simulink model "v2012_PF"  (Simulink 7.6)
(part 4 of 4)

  PQ86 : PMComponent  Tag=PSATblock  Description=Power Flow  PhysicalDomain=psatdomain  LeftPortType=p1  RightPortType=p1  LConnTagsString=__newl0  mask(PQ){p2_3q=[100  115], p4_5q=[0.5061 0.2587]*1.0722*0.0909, p6_7q=[1.2  0.8], p8q=off, p9q=on}
      mask prompts: p2_3q "Power and Voltage Ratings [MVA, kV]"; p4_5q "Active and Reactive Powers [p.u.  p.u.]"; p6_7q "Maximum and Minimum Allowable Voltage [p.u.   p.u.]"; p8q "Allow conversion to impendance for min or max voltage"; p9q "Connected"
      mask help:
      | This block defines a constant power load:
      |
      | P = Pcost.
      | Q = Qcost.
      mask CallbackString: |||fm_block|fm_block
      mask Display: plot([1 -0.5 -0.5 1],[0 0.866 -0.866 0])
  PQ9 : PMComponent  Tag=PSATblock  Description=Power Flow  PhysicalDomain=psatdomain  LeftPortType=p1  RightPortType=p1  LConnTagsString=__newl0  mask(PQ){p2_3q=[100 115], p4_5q=[2.2396 1.0847]*1.0722*0.25, p6_7q=[1.2  0.8], p8q=off, p9q=on}
      mask prompts: p2_3q "Power and Voltage Ratings [MVA, kV]"; p4_5q "Active and Reactive Powers [p.u.  p.u.]"; p6_7q "Maximum and Minimum Allowable Voltage [p.u.   p.u.]"; p8q "Allow conversion to impendance for min or max voltage"; p9q "Connected"
      mask help:
      | This block defines a constant power load:
      |
      | P = Pcost.
      | Q = Qcost.
      mask CallbackString: |||fm_block|fm_block
      mask Display: plot([1 -0.5 -0.5 1],[0 0.866 -0.866 0])
  PQ92 : PMComponent  Tag=PSATblock  Description=Power Flow  PhysicalDomain=psatdomain  LeftPortType=p1  RightPortType=p1  LConnTagsString=__newl0  mask(PQ){p2_3q=[100  115], p4_5q=[0.5061 0.2587]*1.0722*0.0909, p6_7q=[1.2  0.8], p8q=off, p9q=on}
      mask prompts: p2_3q "Power and Voltage Ratings [MVA, kV]"; p4_5q "Active and Reactive Powers [p.u.  p.u.]"; p6_7q "Maximum and Minimum Allowable Voltage [p.u.   p.u.]"; p8q "Allow conversion to impendance for min or max voltage"; p9q "Connected"
      mask help:
      | This block defines a constant power load:
      |
      | P = Pcost.
      | Q = Qcost.
      mask CallbackString: |||fm_block|fm_block
      mask Display: plot([1 -0.5 -0.5 1],[0 0.866 -0.866 0])
  PQ95 : PMComponent  Tag=PSATblock  Description=Power Flow  PhysicalDomain=psatdomain  LeftPortType=p1  RightPortType=p1  LConnTagsString=__newl0  mask(PQ){p2_3q=[100 115], p4_5q=[0.2898 0.2057]*1.0722*0.1667, p6_7q=[1.2  0.8], p8q=off, p9q=on}
      mask prompts: p2_3q "Power and Voltage Ratings [MVA, kV]"; p4_5q "Active and Reactive Powers [p.u.  p.u.]"; p6_7q "Maximum and Minimum Allowable Voltage [p.u.   p.u.]"; p8q "Allow conversion to impendance for min or max voltage"; p9q "Connected"
      mask help:
      | This block defines a constant power load:
      |
      | P = Pcost.
      | Q = Qcost.
      mask CallbackString: |||fm_block|fm_block
      mask Display: plot([1 -0.5 -0.5 1],[0 0.866 -0.866 0])
  PQ96 : PMComponent  Tag=PSATblock  Description=Power Flow  PhysicalDomain=psatdomain  LeftPortType=p1  RightPortType=p1  LConnTagsString=__newl0  mask(PQ){p2_3q=[100 115], p4_5q=[0.2898 0.2057]*1.0722*0.1667, p6_7q=[1.2  0.8], p8q=off, p9q=on}
      mask prompts: p2_3q "Power and Voltage Ratings [MVA, kV]"; p4_5q "Active and Reactive Powers [p.u.  p.u.]"; p6_7q "Maximum and Minimum Allowable Voltage [p.u.   p.u.]"; p8q "Allow conversion to impendance for min or max voltage"; p9q "Connected"
      mask help:
      | This block defines a constant power load:
      |
      | P = Pcost.
      | Q = Qcost.
      mask CallbackString: |||fm_block|fm_block
      mask Display: plot([1 -0.5 -0.5 1],[0 0.866 -0.866 0])
  PQ97 : PMComponent  Tag=PSATblock  Description=Power Flow  PhysicalDomain=psatdomain  LeftPortType=p1  RightPortType=p1  LConnTagsString=__newl0  mask(PQ){p2_3q=[100 115], p4_5q=[0.2898 0.2057]*1.0722*0.1667, p6_7q=[1.2  0.8], p8q=off, p9q=on}
      mask prompts: p2_3q "Power and Voltage Ratings [MVA, kV]"; p4_5q "Active and Reactive Powers [p.u.  p.u.]"; p6_7q "Maximum and Minimum Allowable Voltage [p.u.   p.u.]"; p8q "Allow conversion to impendance for min or max voltage"; p9q "Connected"
      mask help:
      | This block defines a constant power load:
      |
      | P = Pcost.
      | Q = Qcost.
      mask CallbackString: |||fm_block|fm_block
      mask Display: plot([1 -0.5 -0.5 1],[0 0.866 -0.866 0])
  PQ98 : PMComponent  Tag=PSATblock  Description=Power Flow  PhysicalDomain=psatdomain  LeftPortType=p1  RightPortType=p1  LConnTagsString=__newl0  mask(PQ){p2_3q=[100 115], p4_5q=[0.2898 0.2057]*1.0722*0.1667, p6_7q=[1.2  0.8], p8q=off, p9q=on}
      mask prompts: p2_3q "Power and Voltage Ratings [MVA, kV]"; p4_5q "Active and Reactive Powers [p.u.  p.u.]"; p6_7q "Maximum and Minimum Allowable Voltage [p.u.   p.u.]"; p8q "Allow conversion to impendance for min or max voltage"; p9q "Connected"
      mask help:
      | This block defines a constant power load:
      |
      | P = Pcost.
      | Q = Qcost.
      mask CallbackString: |||fm_block|fm_block
      mask Display: plot([1 -0.5 -0.5 1],[0 0.866 -0.866 0])
  PQ99 : PMComponent  Tag=PSATblock  Description=Power Flow  PhysicalDomain=psatdomain  LeftPortType=p1  RightPortType=p1  LConnTagsString=__newl0  mask(PQ){p2_3q=[100 115], p4_5q=[0.2898 0.2057]*1.0722*0.1667, p6_7q=[1.2  0.8], p8q=off, p9q=on}
      mask prompts: p2_3q "Power and Voltage Ratings [MVA, kV]"; p4_5q "Active and Reactive Powers [p.u.  p.u.]"; p6_7q "Maximum and Minimum Allowable Voltage [p.u.   p.u.]"; p8q "Allow conversion to impendance for min or max voltage"; p9q "Connected"
      mask help:
      | This block defines a constant power load:
      |
      | P = Pcost.
      | Q = Qcost.
      mask CallbackString: |||fm_block|fm_block
      mask Display: plot([1 -0.5 -0.5 1],[0 0.866 -0.866 0])
  PV : PMComponent  Tag=PSATblock  Description=Power Flow  PhysicalDomain=psatdomain  LeftPortType=p1  RightPortType=p1  RConnTagsString=__newr0  mask(PV){p2_3q=[100  115], p4q=2.6539+1.75, p5q=1.04, p6_7q=[0.8  -0.2], p8_9q=[1.1  0.9], p10q=1, p11q=on}
      mask prompts: p2_3q "Power and Voltage Ratings [MVA, kV]"; p4q "Active Power [p.u.]"; p5q "Voltage Magnitude [p.u.]"; p6_7q "Qmax and Qmin [p.u.  p.u.]"; p8_9q "Vmax and Vmin [p.u.  p.u.]"; p10q "Loss Participation Factor"; p11q "Connected"
      mask help:
      | This block defines a PV bus for load flow studies:
      |
      | P = Pcost.
      | V = Vdes.
      mask init:
      | [x,y] = fm_draw('circle');
      | [xp,yp] = fm_draw('P');
      mask CallbackString: ||||||fm_block
      mask Display:
      | plot(x,y)
      | color('blue')
      | plot(0.3*xp-0.35,0.6*yp,[0.1 0.3 0.5],[0.3 -0.3 0.3])
  PV1 : PMComponent  Tag=PSATblock  Description=Power Flow  PhysicalDomain=psatdomain  LeftPortType=p1  RightPortType=p1  RConnTagsString=__newr0  mask(PV){p2_3q=[100  115], p4q=5.6441*0.5, p5q=1.04, p6_7q=[0.8  -0.2], p8_9q=[1.1  0.9], p10q=1, p11q=on}
      mask prompts: p2_3q "Power and Voltage Ratings [MVA, kV]"; p4q "Active Power [p.u.]"; p5q "Voltage Magnitude [p.u.]"; p6_7q "Qmax and Qmin [p.u.  p.u.]"; p8_9q "Vmax and Vmin [p.u.  p.u.]"; p10q "Loss Participation Factor"; p11q "Connected"
      mask help:
      | This block defines a PV bus for load flow studies:
      |
      | P = Pcost.
      | V = Vdes.
      mask init:
      | [x,y] = fm_draw('circle');
      | [xp,yp] = fm_draw('P');
      mask CallbackString: ||||||fm_block
      mask Display:
      | plot(x,y)
      | color('blue')
      | plot(0.3*xp-0.35,0.6*yp,[0.1 0.3 0.5],[0.3 -0.3 0.3])
  PV10 : PMComponent  Tag=PSATblock  Description=Power Flow  PhysicalDomain=psatdomain  LeftPortType=p1  RightPortType=p1  RConnTagsString=__newr0  mask(PV){p2_3q=[100  138], p4q=10.4361, p5q=1.04, p6_7q=[0.8  -0.2], p8_9q=[1.1  0.9], p10q=1, p11q=on}
      mask prompts: p2_3q "Power and Voltage Ratings [MVA, kV]"; p4q "Active Power [p.u.]"; p5q "Voltage Magnitude [p.u.]"; p6_7q "Qmax and Qmin [p.u.  p.u.]"; p8_9q "Vmax and Vmin [p.u.  p.u.]"; p10q "Loss Participation Factor"; p11q "Connected"
      mask help:
      | This block defines a PV bus for load flow studies:
      |
      | P = Pcost.
      | V = Vdes.
      mask init:
      | [x,y] = fm_draw('circle');
      | [xp,yp] = fm_draw('P');
      mask CallbackString: ||||||fm_block
      mask Display:
      | plot(x,y)
      | color('blue')
      | plot(0.3*xp-0.35,0.6*yp,[0.1 0.3 0.5],[0.3 -0.3 0.3])
  PV11 : PMComponent  Tag=PSATblock  Description=Power Flow  PhysicalDomain=psatdomain  LeftPortType=p1  RightPortType=p1  RConnTagsString=__newr0  mask(PV){p2_3q=[100  400], p4q=13.1628, p5q=1.03, p6_7q=[0.8  -0.2], p8_9q=[1.1  0.9], p10q=1, p11q=on}
      mask prompts: p2_3q "Power and Voltage Ratings [MVA, kV]"; p4q "Active Power [p.u.]"; p5q "Voltage Magnitude [p.u.]"; p6_7q "Qmax and Qmin [p.u.  p.u.]"; p8_9q "Vmax and Vmin [p.u.  p.u.]"; p10q "Loss Participation Factor"; p11q "Connected"
      mask help:
      | This block defines a PV bus for load flow studies:
      |
      | P = Pcost.
      | V = Vdes.
      mask init:
      | [x,y] = fm_draw('circle');
      | [xp,yp] = fm_draw('P');
      mask CallbackString: ||||||fm_block
      mask Display:
      | plot(x,y)
      | color('blue')
      | plot(0.3*xp-0.35,0.6*yp,[0.1 0.3 0.5],[0.3 -0.3 0.3])
  PV12 : PMComponent  Tag=PSATblock  Description=Power Flow  PhysicalDomain=psatdomain  LeftPortType=p1  RightPortType=p1  RConnTagsString=__newr0  mask(PV){p2_3q=[100  230], p4q=2.9239, p5q=1.03, p6_7q=[0.8  -0.2], p8_9q=[1.1  0.9], p10q=1, p11q=on}
      mask prompts: p2_3q "Power and Voltage Ratings [MVA, kV]"; p4q "Active Power [p.u.]"; p5q "Voltage Magnitude [p.u.]"; p6_7q "Qmax and Qmin [p.u.  p.u.]"; p8_9q "Vmax and Vmin [p.u.  p.u.]"; p10q "Loss Participation Factor"; p11q "Connected"
      mask help:
      | This block defines a PV bus for load flow studies:
      |
      | P = Pcost.
      | V = Vdes.
      mask init:
      | [x,y] = fm_draw('circle');
      | [xp,yp] = fm_draw('P');
      mask CallbackString: ||||||fm_block
      mask Display:
      | plot(x,y)
      | color('blue')
      | plot(0.3*xp-0.35,0.6*yp,[0.1 0.3 0.5],[0.3 -0.3 0.3])
  PV13 : PMComponent  Tag=PSATblock  Description=Power Flow  PhysicalDomain=psatdomain  LeftPortType=p1  RightPortType=p1  RConnTagsString=__newr0  mask(PV){p2_3q=[100  230], p4q=2.1010+2.8, p5q=1.04, p6_7q=[0.8  -0.2], p8_9q=[1.1  0.9], p10q=1, p11q=on}
      mask prompts: p2_3q "Power and Voltage Ratings [MVA, kV]"; p4q "Active Power [p.u.]"; p5q "Voltage Magnitude [p.u.]"; p6_7q "Qmax and Qmin [p.u.  p.u.]"; p8_9q "Vmax and Vmin [p.u.  p.u.]"; p10q "Loss Participation Factor"; p11q "Connected"
      mask help:
      | This block defines a PV bus for load flow studies:
      |
      | P = Pcost.
      | V = Vdes.
      mask init:
      | [x,y] = fm_draw('circle');
      | [xp,yp] = fm_draw('P');
      mask CallbackString: ||||||fm_block
      mask Display:
      | plot(x,y)
      | color('blue')
      | plot(0.3*xp-0.35,0.6*yp,[0.1 0.3 0.5],[0.3 -0.3 0.3])
  PV14 : PMComponent  Tag=PSATblock  Description=Power Flow  PhysicalDomain=psatdomain  LeftPortType=p1  RightPortType=p1  RConnTagsString=__newr0  mask(PV){p2_3q=[100  400], p4q=14.6386, p5q=1.03, p6_7q=[0.8  -0.2], p8_9q=[1.1  0.9], p10q=1, p11q=on}
      mask prompts: p2_3q "Power and Voltage Ratings [MVA, kV]"; p4q "Active Power [p.u.]"; p5q "Voltage Magnitude [p.u.]"; p6_7q "Qmax and Qmin [p.u.  p.u.]"; p8_9q "Vmax and Vmin [p.u.  p.u.]"; p10q "Loss Participation Factor"; p11q "Connected"
      mask help:
      | This block defines a PV bus for load flow studies:
      |
      | P = Pcost.
      | V = Vdes.
      mask init:
      | [x,y] = fm_draw('circle');
      | [xp,yp] = fm_draw('P');
      mask CallbackString: ||||||fm_block
      mask Display:
      | plot(x,y)
      | color('blue')
      | plot(0.3*xp-0.35,0.6*yp,[0.1 0.3 0.5],[0.3 -0.3 0.3])
  PV15 : PMComponent  Tag=PSATblock  Description=Power Flow  PhysicalDomain=psatdomain  LeftPortType=p1  RightPortType=p1  RConnTagsString=__newr0  mask(PV){p2_3q=[100  230], p4q=5.04, p5q=1.02, p6_7q=[0.8  -0.2], p8_9q=[1.1  0.9], p10q=1, p11q=on}
      mask prompts: p2_3q "Power and Voltage Ratings [MVA, kV]"; p4q "Active Power [p.u.]"; p5q "Voltage Magnitude [p.u.]"; p6_7q "Qmax and Qmin [p.u.  p.u.]"; p8_9q "Vmax and Vmin [p.u.  p.u.]"; p10q "Loss Participation Factor"; p11q "Connected"
      mask help:
      | This block defines a PV bus for load flow studies:
      |
      | P = Pcost.
      | V = Vdes.
      mask init:
      | [x,y] = fm_draw('circle');
      | [xp,yp] = fm_draw('P');
      mask CallbackString: ||||||fm_block
      mask Display:
      | plot(x,y)
      | color('blue')
      | plot(0.3*xp-0.35,0.6*yp,[0.1 0.3 0.5],[0.3 -0.3 0.3])
  PV16 : PMComponent  Tag=PSATblock  Description=Power Flow  PhysicalDomain=psatdomain  LeftPortType=p1  RightPortType=p1  RConnTagsString=__newr0  mask(PV){p2_3q=[100  400], p4q=4.2*0.5, p5q=1.02, p6_7q=[0.8  -0.2], p8_9q=[1.1  0.9], p10q=1, p11q=on}
      mask prompts: p2_3q "Power and Voltage Ratings [MVA, kV]"; p4q "Active Power [p.u.]"; p5q "Voltage Magnitude [p.u.]"; p6_7q "Qmax and Qmin [p.u.  p.u.]"; p8_9q "Vmax and Vmin [p.u.  p.u.]"; p10q "Loss Participation Factor"; p11q "Connected"
      mask help:
      | This block defines a PV bus for load flow studies:
      |
      | P = Pcost.
      | V = Vdes.
      mask init:
      | [x,y] = fm_draw('circle');
      | [xp,yp] = fm_draw('P');
      mask CallbackString: ||||||fm_block
      mask Display:
      | plot(x,y)
      | color('blue')
      | plot(0.3*xp-0.35,0.6*yp,[0.1 0.3 0.5],[0.3 -0.3 0.3])
  PV17 : PMComponent  Tag=PSATblock  Description=Power Flow  PhysicalDomain=psatdomain  LeftPortType=p1  RightPortType=p1  RConnTagsString=__newr0  mask(PV){p2_3q=[100  400], p4q=4.2*0.5, p5q=1.02, p6_7q=[0.8  -0.2], p8_9q=[1.1  0.9], p10q=1, p11q=on}
      mask prompts: p2_3q "Power and Voltage Ratings [MVA, kV]"; p4q "Active Power [p.u.]"; p5q "Voltage Magnitude [p.u.]"; p6_7q "Qmax and Qmin [p.u.  p.u.]"; p8_9q "Vmax and Vmin [p.u.  p.u.]"; p10q "Loss Participation Factor"; p11q "Connected"
      mask help:
      | This block defines a PV bus for load flow studies:
      |
      | P = Pcost.
      | V = Vdes.
      mask init:
      | [x,y] = fm_draw('circle');
      | [xp,yp] = fm_draw('P');
      mask CallbackString: ||||||fm_block
      mask Display:
      | plot(x,y)
      | color('blue')
      | plot(0.3*xp-0.35,0.6*yp,[0.1 0.3 0.5],[0.3 -0.3 0.3])
  PV18 : PMComponent  Tag=PSATblock  Description=Power Flow  PhysicalDomain=psatdomain  LeftPortType=p1  RightPortType=p1  RConnTagsString=__newr0  mask(PV){p2_3q=[100  230], p4q=1.05, p5q=1.02, p6_7q=[0.8  -0.2], p8_9q=[1.1  0.9], p10q=1, p11q=on}
      mask prompts: p2_3q "Power and Voltage Ratings [MVA, kV]"; p4q "Active Power [p.u.]"; p5q "Voltage Magnitude [p.u.]"; p6_7q "Qmax and Qmin [p.u.  p.u.]"; p8_9q "Vmax and Vmin [p.u.  p.u.]"; p10q "Loss Participation Factor"; p11q "Connected"
      mask help:
      | This block defines a PV bus for load flow studies:
      |
      | P = Pcost.
      | V = Vdes.
      mask init:
      | [x,y] = fm_draw('circle');
      | [xp,yp] = fm_draw('P');
      mask CallbackString: ||||||fm_block
      mask Display:
      | plot(x,y)
      | color('blue')
      | plot(0.3*xp-0.35,0.6*yp,[0.1 0.3 0.5],[0.3 -0.3 0.3])
  PV19 : PMComponent  Tag=PSATblock  Description=Power Flow  PhysicalDomain=psatdomain  LeftPortType=p1  RightPortType=p1  RConnTagsString=__newr0  mask(PV){p2_3q=[100  230], p4q=2.997*0.5, p5q=1.02, p6_7q=[0.8  -0.2], p8_9q=[1.1  0.9], p10q=1, p11q=on}
      mask prompts: p2_3q "Power and Voltage Ratings [MVA, kV]"; p4q "Active Power [p.u.]"; p5q "Voltage Magnitude [p.u.]"; p6_7q "Qmax and Qmin [p.u.  p.u.]"; p8_9q "Vmax and Vmin [p.u.  p.u.]"; p10q "Loss Participation Factor"; p11q "Connected"
      mask help:
      | This block defines a PV bus for load flow studies:
      |
      | P = Pcost.
      | V = Vdes.
      mask init:
      | [x,y] = fm_draw('circle');
      | [xp,yp] = fm_draw('P');
      mask CallbackString: ||||||fm_block
      mask Display:
      | plot(x,y)
      | color('blue')
      | plot(0.3*xp-0.35,0.6*yp,[0.1 0.3 0.5],[0.3 -0.3 0.3])
  PV2 : PMComponent  Tag=PSATblock  Description=Power Flow  PhysicalDomain=psatdomain  LeftPortType=p1  RightPortType=p1  RConnTagsString=__newr0  mask(PV){p2_3q=[100  230], p4q=11.1020, p5q=1.04, p6_7q=[0.8  -0.2], p8_9q=[1.1  0.9], p10q=1, p11q=on}
      mask prompts: p2_3q "Power and Voltage Ratings [MVA, kV]"; p4q "Active Power [p.u.]"; p5q "Voltage Magnitude [p.u.]"; p6_7q "Qmax and Qmin [p.u.  p.u.]"; p8_9q "Vmax and Vmin [p.u.  p.u.]"; p10q "Loss Participation Factor"; p11q "Connected"
      mask help:
      | This block defines a PV bus for load flow studies:
      |
      | P = Pcost.
      | V = Vdes.
      mask init:
      | [x,y] = fm_draw('circle');
      | [xp,yp] = fm_draw('P');
      mask CallbackString: ||||||fm_block
      mask Display:
      | plot(x,y)
      | color('blue')
      | plot(0.3*xp-0.35,0.6*yp,[0.1 0.3 0.5],[0.3 -0.3 0.3])
  PV20 : PMComponent  Tag=PSATblock  Description=Power Flow  PhysicalDomain=psatdomain  LeftPortType=p1  RightPortType=p1  RConnTagsString=__newr0  mask(PV){p2_3q=[100  230], p4q=7.77, p5q=1.04, p6_7q=[0.8  -0.2], p8_9q=[1.1  0.9], p10q=1, p11q=on}
      mask prompts: p2_3q "Power and Voltage Ratings [MVA, kV]"; p4q "Active Power [p.u.]"; p5q "Voltage Magnitude [p.u.]"; p6_7q "Qmax and Qmin [p.u.  p.u.]"; p8_9q "Vmax and Vmin [p.u.  p.u.]"; p10q "Loss Participation Factor"; p11q "Connected"
      mask help:
      | This block defines a PV bus for load flow studies:
      |
      | P = Pcost.
      | V = Vdes.
      mask init:
      | [x,y] = fm_draw('circle');
      | [xp,yp] = fm_draw('P');
      mask CallbackString: ||||||fm_block
      mask Display:
      | plot(x,y)
      | color('blue')
      | plot(0.3*xp-0.35,0.6*yp,[0.1 0.3 0.5],[0.3 -0.3 0.3])
  PV21 : PMComponent  Tag=PSATblock  Description=Power Flow  PhysicalDomain=psatdomain  LeftPortType=p1  RightPortType=p1  RConnTagsString=__newr0  mask(PV){p2_3q=[100  115], p4q=0.4795, p5q=1.02, p6_7q=[0.8  -0.2], p8_9q=[1.1  0.9], p10q=1, p11q=on}
      mask prompts: p2_3q "Power and Voltage Ratings [MVA, kV]"; p4q "Active Power [p.u.]"; p5q "Voltage Magnitude [p.u.]"; p6_7q "Qmax and Qmin [p.u.  p.u.]"; p8_9q "Vmax and Vmin [p.u.  p.u.]"; p10q "Loss Participation Factor"; p11q "Connected"
      mask help:
      | This block defines a PV bus for load flow studies:
      |
      | P = Pcost.
      | V = Vdes.
      mask init:
      | [x,y] = fm_draw('circle');
      | [xp,yp] = fm_draw('P');
      mask CallbackString: ||||||fm_block
      mask Display:
      | plot(x,y)
      | color('blue')
      | plot(0.3*xp-0.35,0.6*yp,[0.1 0.3 0.5],[0.3 -0.3 0.3])
  PV22 : PMComponent  Tag=PSATblock  Description=Power Flow  PhysicalDomain=psatdomain  LeftPortType=p1  RightPortType=p1  RConnTagsString=__newr0  mask(PV){p2_3q=[100  230], p4q=1.1667, p5q=1.02, p6_7q=[0.8  -0.2], p8_9q=[1.1  0.9], p10q=1, p11q=on}
      mask prompts: p2_3q "Power and Voltage Ratings [MVA, kV]"; p4q "Active Power [p.u.]"; p5q "Voltage Magnitude [p.u.]"; p6_7q "Qmax and Qmin [p.u.  p.u.]"; p8_9q "Vmax and Vmin [p.u.  p.u.]"; p10q "Loss Participation Factor"; p11q "Connected"
      mask help:
      | This block defines a PV bus for load flow studies:
      |
      | P = Pcost.
      | V = Vdes.
      mask init:
      | [x,y] = fm_draw('circle');
      | [xp,yp] = fm_draw('P');
      mask CallbackString: ||||||fm_block
      mask Display:
      | plot(x,y)
      | color('blue')
      | plot(0.3*xp-0.35,0.6*yp,[0.1 0.3 0.5],[0.3 -0.3 0.3])
  PV23 : PMComponent  Tag=PSATblock  Description=Power Flow  PhysicalDomain=psatdomain  LeftPortType=p1  RightPortType=p1  RConnTagsString=__newr0  mask(PV){p2_3q=[100  115], p4q=4.2029*0.1, p5q=0.9833, p6_7q=[0.8  -0.2], p8_9q=[1.1  0.9], p10q=1, p11q=on}
      mask prompts: p2_3q "Power and Voltage Ratings [MVA, kV]"; p4q "Active Power [p.u.]"; p5q "Voltage Magnitude [p.u.]"; p6_7q "Qmax and Qmin [p.u.  p.u.]"; p8_9q "Vmax and Vmin [p.u.  p.u.]"; p10q "Loss Participation Factor"; p11q "Connected"
      mask help:
      | This block defines a PV bus for load flow studies:
      |
      | P = Pcost.
      | V = Vdes.
      mask init:
      | [x,y] = fm_draw('circle');
      | [xp,yp] = fm_draw('P');
      mask CallbackString: ||||||fm_block
      mask Display:
      | plot(x,y)
      | color('blue')
      | plot(0.3*xp-0.35,0.6*yp,[0.1 0.3 0.5],[0.3 -0.3 0.3])
  PV24 : PMComponent  Tag=PSATblock  Description=Power Flow  PhysicalDomain=psatdomain  LeftPortType=p1  RightPortType=p1  RConnTagsString=__newr0  mask(PV){p2_3q=[100  115], p4q=0.07, p5q=1.02, p6_7q=[0.8  -0.2], p8_9q=[1.1  0.9], p10q=1, p11q=on}
      mask prompts: p2_3q "Power and Voltage Ratings [MVA, kV]"; p4q "Active Power [p.u.]"; p5q "Voltage Magnitude [p.u.]"; p6_7q "Qmax and Qmin [p.u.  p.u.]"; p8_9q "Vmax and Vmin [p.u.  p.u.]"; p10q "Loss Participation Factor"; p11q "Connected"
      mask help:
      | This block defines a PV bus for load flow studies:
      |
      | P = Pcost.
      | V = Vdes.
      mask init:
      | [x,y] = fm_draw('circle');
      | [xp,yp] = fm_draw('P');
      mask CallbackString: ||||||fm_block
      mask Display:
      | plot(x,y)
      | color('blue')
      | plot(0.3*xp-0.35,0.6*yp,[0.1 0.3 0.5],[0.3 -0.3 0.3])
  PV25 : PMComponent  Tag=PSATblock  Description=Power Flow  PhysicalDomain=psatdomain  LeftPortType=p1  RightPortType=p1  RConnTagsString=__newr0  mask(PV){p2_3q=[100  115], p4q=2.8610*0.5, p5q=1.04, p6_7q=[0.8  -0.2], p8_9q=[1.1  0.9], p10q=1, p11q=on}
      mask prompts: p2_3q "Power and Voltage Ratings [MVA, kV]"; p4q "Active Power [p.u.]"; p5q "Voltage Magnitude [p.u.]"; p6_7q "Qmax and Qmin [p.u.  p.u.]"; p8_9q "Vmax and Vmin [p.u.  p.u.]"; p10q "Loss Participation Factor"; p11q "Connected"
      mask help:
      | This block defines a PV bus for load flow studies:
      |
      | P = Pcost.
      | V = Vdes.
      mask init:
      | [x,y] = fm_draw('circle');
      | [xp,yp] = fm_draw('P');
      mask CallbackString: ||||||fm_block
      mask Display:
      | plot(x,y)
      | color('blue')
      | plot(0.3*xp-0.35,0.6*yp,[0.1 0.3 0.5],[0.3 -0.3 0.3])
  PV26 : PMComponent  Tag=PSATblock  Description=Power Flow  PhysicalDomain=psatdomain  LeftPortType=p1  RightPortType=p1  RConnTagsString=__newr0  mask(PV){p2_3q=[100  115], p4q=0.6832, p5q=1.04, p6_7q=[0.8  -0.2], p8_9q=[1.1  0.9], p10q=1, p11q=on}
      mask prompts: p2_3q "Power and Voltage Ratings [MVA, kV]"; p4q "Active Power [p.u.]"; p5q "Voltage Magnitude [p.u.]"; p6_7q "Qmax and Qmin [p.u.  p.u.]"; p8_9q "Vmax and Vmin [p.u.  p.u.]"; p10q "Loss Participation Factor"; p11q "Connected"
      mask help:
      | This block defines a PV bus for load flow studies:
      |
      | P = Pcost.
      | V = Vdes.
      mask init:
      | [x,y] = fm_draw('circle');
      | [xp,yp] = fm_draw('P');
      mask CallbackString: ||||||fm_block
      mask Display:
      | plot(x,y)
      | color('blue')
      | plot(0.3*xp-0.35,0.6*yp,[0.1 0.3 0.5],[0.3 -0.3 0.3])
  PV27 : PMComponent  Tag=PSATblock  Description=Power Flow  PhysicalDomain=psatdomain  LeftPortType=p1  RightPortType=p1  RConnTagsString=__newr0  mask(PV){p2_3q=[100  115], p4q=1.8298, p5q=1.02, p6_7q=[0.8  -0.2], p8_9q=[1.1  0.9], p10q=1, p11q=on}
      mask prompts: p2_3q "Power and Voltage Ratings [MVA, kV]"; p4q "Active Power [p.u.]"; p5q "Voltage Magnitude [p.u.]"; p6_7q "Qmax and Qmin [p.u.  p.u.]"; p8_9q "Vmax and Vmin [p.u.  p.u.]"; p10q "Loss Participation Factor"; p11q "Connected"
      mask help:
      | This block defines a PV bus for load flow studies:
      |
      | P = Pcost.
      | V = Vdes.
      mask init:
      | [x,y] = fm_draw('circle');
      | [xp,yp] = fm_draw('P');
      mask CallbackString: ||||||fm_block
      mask Display:
      | plot(x,y)
      | color('blue')
      | plot(0.3*xp-0.35,0.6*yp,[0.1 0.3 0.5],[0.3 -0.3 0.3])
  PV28 : PMComponent  Tag=PSATblock  Description=Power Flow  PhysicalDomain=psatdomain  LeftPortType=p1  RightPortType=p1  RConnTagsString=__newr0  mask(PV){p2_3q=[100  115], p4q=4.1668*0.1, p5q=0.9513, p6_7q=[0.8  -0.2], p8_9q=[1.1  0.9], p10q=1, p11q=on}
      mask prompts: p2_3q "Power and Voltage Ratings [MVA, kV]"; p4q "Active Power [p.u.]"; p5q "Voltage Magnitude [p.u.]"; p6_7q "Qmax and Qmin [p.u.  p.u.]"; p8_9q "Vmax and Vmin [p.u.  p.u.]"; p10q "Loss Participation Factor"; p11q "Connected"
      mask help:
      | This block defines a PV bus for load flow studies:
      |
      | P = Pcost.
      | V = Vdes.
      mask init:
      | [x,y] = fm_draw('circle');
      | [xp,yp] = fm_draw('P');
      mask CallbackString: ||||||fm_block
      mask Display:
      | plot(x,y)
      | color('blue')
      | plot(0.3*xp-0.35,0.6*yp,[0.1 0.3 0.5],[0.3 -0.3 0.3])
  PV29 : PMComponent  Tag=PSATblock  Description=Power Flow  PhysicalDomain=psatdomain  LeftPortType=p1  RightPortType=p1  RConnTagsString=__newr0  mask(PV){p2_3q=[100  115], p4q=0.1499, p5q=1.02, p6_7q=[0.8  -0.2], p8_9q=[1.1  0.9], p10q=1, p11q=on}
      mask prompts: p2_3q "Power and Voltage Ratings [MVA, kV]"; p4q "Active Power [p.u.]"; p5q "Voltage Magnitude [p.u.]"; p6_7q "Qmax and Qmin [p.u.  p.u.]"; p8_9q "Vmax and Vmin [p.u.  p.u.]"; p10q "Loss Participation Factor"; p11q "Connected"
      mask help:
      | This block defines a PV bus for load flow studies:
      |
      | P = Pcost.
      | V = Vdes.
      mask init:
      | [x,y] = fm_draw('circle');
      | [xp,yp] = fm_draw('P');
      mask CallbackString: ||||||fm_block
      mask Display:
      | plot(x,y)
      | color('blue')
      | plot(0.3*xp-0.35,0.6*yp,[0.1 0.3 0.5],[0.3 -0.3 0.3])
  PV3 : PMComponent  Tag=PSATblock  Description=Power Flow  PhysicalDomain=psatdomain  LeftPortType=p1  RightPortType=p1  RConnTagsString=__newr0  mask(PV){p2_3q=[100  230], p4q=2.8610*0.5, p5q=1.04, p6_7q=[0.8  -0.2], p8_9q=[1.1  0.9], p10q=1, p11q=on}
      mask prompts: p2_3q "Power and Voltage Ratings [MVA, kV]"; p4q "Active Power [p.u.]"; p5q "Voltage Magnitude [p.u.]"; p6_7q "Qmax and Qmin [p.u.  p.u.]"; p8_9q "Vmax and Vmin [p.u.  p.u.]"; p10q "Loss Participation Factor"; p11q "Connected"
      mask help:
      | This block defines a PV bus for load flow studies:
      |
      | P = Pcost.
      | V = Vdes.
      mask init:
      | [x,y] = fm_draw('circle');
      | [xp,yp] = fm_draw('P');
      mask CallbackString: ||||||fm_block
      mask Display:
      | plot(x,y)
      | color('blue')
      | plot(0.3*xp-0.35,0.6*yp,[0.1 0.3 0.5],[0.3 -0.3 0.3])
  PV30 : PMComponent  Tag=PSATblock  Description=Power Flow  PhysicalDomain=psatdomain  LeftPortType=p1  RightPortType=p1  RConnTagsString=__newr0  mask(PV){p2_3q=[100  115], p4q=0.28, p5q=1.02, p6_7q=[0.8  -0.2], p8_9q=[1.1  0.9], p10q=1, p11q=on}
      mask prompts: p2_3q "Power and Voltage Ratings [MVA, kV]"; p4q "Active Power [p.u.]"; p5q "Voltage Magnitude [p.u.]"; p6_7q "Qmax and Qmin [p.u.  p.u.]"; p8_9q "Vmax and Vmin [p.u.  p.u.]"; p10q "Loss Participation Factor"; p11q "Connected"
      mask help:
      | This block defines a PV bus for load flow studies:
      |
      | P = Pcost.
      | V = Vdes.
      mask init:
      | [x,y] = fm_draw('circle');
      | [xp,yp] = fm_draw('P');
      mask CallbackString: ||||||fm_block
      mask Display:
      | plot(x,y)
      | color('blue')
      | plot(0.3*xp-0.35,0.6*yp,[0.1 0.3 0.5],[0.3 -0.3 0.3])
  PV38 : PMComponent  Tag=PSATblock  Description=Power Flow  PhysicalDomain=psatdomain  LeftPortType=p1  RightPortType=p1  RConnTagsString=__newr0  mask(PV){p2_3q=[100  115], p4q=5.6441*0.5, p5q=1.04, p6_7q=[0.8  -0.2], p8_9q=[1.1  0.9], p10q=1, p11q=on}
      mask prompts: p2_3q "Power and Voltage Ratings [MVA, kV]"; p4q "Active Power [p.u.]"; p5q "Voltage Magnitude [p.u.]"; p6_7q "Qmax and Qmin [p.u.  p.u.]"; p8_9q "Vmax and Vmin [p.u.  p.u.]"; p10q "Loss Participation Factor"; p11q "Connected"
      mask help:
      | This block defines a PV bus for load flow studies:
      |
      | P = Pcost.
      | V = Vdes.
      mask init:
      | [x,y] = fm_draw('circle');
      | [xp,yp] = fm_draw('P');
      mask CallbackString: ||||||fm_block
      mask Display:
      | plot(x,y)
      | color('blue')
      | plot(0.3*xp-0.35,0.6*yp,[0.1 0.3 0.5],[0.3 -0.3 0.3])
  PV4 : PMComponent  Tag=PSATblock  Description=Power Flow  PhysicalDomain=psatdomain  LeftPortType=p1  RightPortType=p1  RConnTagsString=__newr0  mask(PV){p2_3q=[100  230], p4q=1.7982, p5q=1.02, p6_7q=[0.8  -0.2], p8_9q=[1.1  0.9], p10q=1, p11q=on}
      mask prompts: p2_3q "Power and Voltage Ratings [MVA, kV]"; p4q "Active Power [p.u.]"; p5q "Voltage Magnitude [p.u.]"; p6_7q "Qmax and Qmin [p.u.  p.u.]"; p8_9q "Vmax and Vmin [p.u.  p.u.]"; p10q "Loss Participation Factor"; p11q "Connected"
      mask help:
      | This block defines a PV bus for load flow studies:
      |
      | P = Pcost.
      | V = Vdes.
      mask init:
      | [x,y] = fm_draw('circle');
      | [xp,yp] = fm_draw('P');
      mask CallbackString: ||||||fm_block
      mask Display:
      | plot(x,y)
      | color('blue')
      | plot(0.3*xp-0.35,0.6*yp,[0.1 0.3 0.5],[0.3 -0.3 0.3])
  PV5 : PMComponent  Tag=PSATblock  Description=Power Flow  PhysicalDomain=psatdomain  LeftPortType=p1  RightPortType=p1  RConnTagsString=__newr0  mask(PV){p2_3q=[100  138], p4q=4.62, p5q=1.04, p6_7q=[0.8  -0.2], p8_9q=[1.1  0.9], p10q=1, p11q=on}
      mask prompts: p2_3q "Power and Voltage Ratings [MVA, kV]"; p4q "Active Power [p.u.]"; p5q "Voltage Magnitude [p.u.]"; p6_7q "Qmax and Qmin [p.u.  p.u.]"; p8_9q "Vmax and Vmin [p.u.  p.u.]"; p10q "Loss Participation Factor"; p11q "Connected"
      mask help:
      | This block defines a PV bus for load flow studies:
      |
      | P = Pcost.
      | V = Vdes.
      mask init:
      | [x,y] = fm_draw('circle');
      | [xp,yp] = fm_draw('P');
      mask CallbackString: ||||||fm_block
      mask Display:
      | plot(x,y)
      | color('blue')
      | plot(0.3*xp-0.35,0.6*yp,[0.1 0.3 0.5],[0.3 -0.3 0.3])
  PV6 : PMComponent  Tag=PSATblock  Description=Power Flow  PhysicalDomain=psatdomain  LeftPortType=p1  RightPortType=p1  RConnTagsString=__newr0  mask(PV){p2_3q=[100  230], p4q=2.6539+4.83, p5q=1.02, p6_7q=[0.8  -0.2], p8_9q=[1.1  0.9], p10q=1, p11q=on}
      mask prompts: p2_3q "Power and Voltage Ratings [MVA, kV]"; p4q "Active Power [p.u.]"; p5q "Voltage Magnitude [p.u.]"; p6_7q "Qmax and Qmin [p.u.  p.u.]"; p8_9q "Vmax and Vmin [p.u.  p.u.]"; p10q "Loss Participation Factor"; p11q "Connected"
      mask help:
      | This block defines a PV bus for load flow studies:
      |
      | P = Pcost.
      | V = Vdes.
      mask init:
      | [x,y] = fm_draw('circle');
      | [xp,yp] = fm_draw('P');
      mask CallbackString: ||||||fm_block
      mask Display:
      | plot(x,y)
      | color('blue')
      | plot(0.3*xp-0.35,0.6*yp,[0.1 0.3 0.5],[0.3 -0.3 0.3])
  PV7 : PMComponent  Tag=PSATblock  Description=Power Flow  PhysicalDomain=psatdomain  LeftPortType=p1  RightPortType=p1  RConnTagsString=__newr0  mask(PV){p2_3q=[100  400], p4q=11.7691, p5q=1.04, p6_7q=[0.8  -0.2], p8_9q=[1.1  0.9], p10q=1, p11q=on}
      mask prompts: p2_3q "Power and Voltage Ratings [MVA, kV]"; p4q "Active Power [p.u.]"; p5q "Voltage Magnitude [p.u.]"; p6_7q "Qmax and Qmin [p.u.  p.u.]"; p8_9q "Vmax and Vmin [p.u.  p.u.]"; p10q "Loss Participation Factor"; p11q "Connected"
      mask help:
      | This block defines a PV bus for load flow studies:
      |
      | P = Pcost.
      | V = Vdes.
      mask init:
      | [x,y] = fm_draw('circle');
      | [xp,yp] = fm_draw('P');
      mask CallbackString: ||||||fm_block
      mask Display:
      | plot(x,y)
      | color('blue')
      | plot(0.3*xp-0.35,0.6*yp,[0.1 0.3 0.5],[0.3 -0.3 0.3])
  PV8 : PMComponent  Tag=PSATblock  Description=Power Flow  PhysicalDomain=psatdomain  LeftPortType=p1  RightPortType=p1  RConnTagsString=__newr0  mask(PV){p2_3q=[100  230], p4q=3.2368, p5q=1.04, p6_7q=[0.8  -0.2], p8_9q=[1.1  0.9], p10q=1, p11q=on}
      mask prompts: p2_3q "Power and Voltage Ratings [MVA, kV]"; p4q "Active Power [p.u.]"; p5q "Voltage Magnitude [p.u.]"; p6_7q "Qmax and Qmin [p.u.  p.u.]"; p8_9q "Vmax and Vmin [p.u.  p.u.]"; p10q "Loss Participation Factor"; p11q "Connected"
      mask help:
      | This block defines a PV bus for load flow studies:
      |
      | P = Pcost.
      | V = Vdes.
      mask init:
      | [x,y] = fm_draw('circle');
      | [xp,yp] = fm_draw('P');
      mask CallbackString: ||||||fm_block
      mask Display:
      | plot(x,y)
      | color('blue')
      | plot(0.3*xp-0.35,0.6*yp,[0.1 0.3 0.5],[0.3 -0.3 0.3])
  PV9 : PMComponent  Tag=PSATblock  Description=Power Flow  PhysicalDomain=psatdomain  LeftPortType=p1  RightPortType=p1  RConnTagsString=__newr0  mask(PV){p2_3q=[100  400], p4q=13.5944, p5q=1.04, p6_7q=[0.8  -0.2], p8_9q=[1.1  0.9], p10q=1, p11q=on}
      mask prompts: p2_3q "Power and Voltage Ratings [MVA, kV]"; p4q "Active Power [p.u.]"; p5q "Voltage Magnitude [p.u.]"; p6_7q "Qmax and Qmin [p.u.  p.u.]"; p8_9q "Vmax and Vmin [p.u.  p.u.]"; p10q "Loss Participation Factor"; p11q "Connected"
      mask help:
      | This block defines a PV bus for load flow studies:
      |
      | P = Pcost.
      | V = Vdes.
      mask init:
      | [x,y] = fm_draw('circle');
      | [xp,yp] = fm_draw('P');
      mask CallbackString: ||||||fm_block
      mask Display:
      | plot(x,y)
      | color('blue')
      | plot(0.3*xp-0.35,0.6*yp,[0.1 0.3 0.5],[0.3 -0.3 0.3])
  Palital 400kV : PMComponent  Tag=PSATblock  Description=Connection  PhysicalDomain=psatdomain  LeftPortType=p1  RightPortType=p1  LConnTagsString=__newl0|__newl1|__newl2  RConnTagsString=__newr0|__newr1  mask(Bus){in=3, out=2, p2q=400, p3_4q=[1.0189    -0.15846], p5q=1, p6q=1}
      mask prompts: in "Number of inputs:"; out "Number of outputs:"; p2q "Voltage Rating [kV]"; p3_4q "Voltage initial guess [p.u.  rad]"; p5q "Area number"; p6q "Region number"
      mask help: Bus block.
      mask init:
      | fm_inout
      settings: AttributesFormatString="|V| =  1.0017 p.u.\\n<V  = -0.1078 rad"
      mask CallbackString: ||||fm_block|
      mask Display: plot([0 1 1 0 0],[0 0 1 1 0])
  Palo Grande : PMComponent  Tag=PSATblock  Description=Connection  PhysicalDomain=psatdomain  LeftPortType=p1  RightPortType=p1  LConnTagsString=__newl0  RConnTagsString=__newr0|__newr1  mask(Bus){in=1, out=2, p2q=115, p3_4q=[1.0023    -0.25717], p5q=1, p6q=1}
      mask prompts: in "Number of inputs:"; out "Number of outputs:"; p2q "Voltage Rating [kV]"; p3_4q "Voltage initial guess [p.u.  rad]"; p5q "Area number"; p6q "Region number"
      mask help: Bus block.
      mask init:
      | fm_inout
      settings: AttributesFormatString="|V| =  1.0139 p.u.\\n<V  =  0.4686 rad"
      mask CallbackString: ||||fm_block|
      mask Display: plot([0 1 1 0 0],[0 0 1 1 0])
  Papelon 230kV : PMComponent  Tag=PSATblock  Description=Connection  PhysicalDomain=psatdomain  LeftPortType=p1  RightPortType=p1  LConnTagsString=__newl0|__newl1  RConnTagsString=__newr0|__newr1|__newr2  mask(Bus){in=2, out=3, p2q=230, p3_4q=[0.99933     -0.4575], p5q=1, p6q=1}
      mask prompts: in "Number of inputs:"; out "Number of outputs:"; p2q "Voltage Rating [kV]"; p3_4q "Voltage initial guess [p.u.  rad]"; p5q "Area number"; p6q "Region number"
      mask help: Bus block.
      mask init:
      | fm_inout
      settings: AttributesFormatString="|V| =  1.0156 p.u.\\n<V  = -0.1966 rad"
      mask CallbackString: ||||fm_block|
      mask Display: plot([0 1 1 0 0],[0 0 1 1 0])
  Pena Larga : PMComponent  Tag=PSATblock  Description=Connection  PhysicalDomain=psatdomain  LeftPortType=p1  RightPortType=p1  LConnTagsString=__newl0|__newl1  RConnTagsString=__newr0  mask(Bus){in=2, out=1, p2q=115, p3_4q=[1.0023    -0.25717], p5q=1, p6q=1}
      mask prompts: in "Number of inputs:"; out "Number of outputs:"; p2q "Voltage Rating [kV]"; p3_4q "Voltage initial guess [p.u.  rad]"; p5q "Area number"; p6q "Region number"
      mask help: Bus block.
      mask init:
      | fm_inout
      settings: AttributesFormatString="|V| =  1.02   p.u.\\n<V  =  0.1072 rad"
      mask CallbackString: ||||fm_block|
      mask Display: plot([0 1 1 0 0],[0 0 1 1 0])
  Peonias : PMComponent  Tag=PSATblock  Description=Connection  PhysicalDomain=psatdomain  LeftPortType=p1  RightPortType=p1  LConnTagsString=__newl0|__newl1  RConnTagsString=__newr0|__newr1  mask(Bus){in=2, out=2, p2q=230, p3_4q=[0.98842    -0.82663], p5q=1, p6q=1}
      mask prompts: in "Number of inputs:"; out "Number of outputs:"; p2q "Voltage Rating [kV]"; p3_4q "Voltage initial guess [p.u.  rad]"; p5q "Area number"; p6q "Region number"
      mask help: Bus block.
      mask init:
      | fm_inout
      settings: AttributesFormatString="|V| =  1.0313 p.u.\\n<V  = -0.0293 rad"
      mask CallbackString: ||||fm_block|
      mask Display: plot([0 1 1 0 0],[0 0 1 1 0])
  Planta Centro 230kV : PMComponent  Tag=PSATblock  Description=Connection  PhysicalDomain=psatdomain  LeftPortType=p1  RightPortType=p1  LConnTagsString=__newl0|__newl1  RConnTagsString=__newr0|__newr1|__newr2|__newr3|__newr4|__newr5  mask(Bus){in=2, out=6, p2q=230, p3_4q=[0.99115    -0.50302], p5q=1, p6q=1}
      mask prompts: in "Number of inputs:"; out "Number of outputs:"; p2q "Voltage Rating [kV]"; p3_4q "Voltage initial guess [p.u.  rad]"; p5q "Area number"; p6q "Region number"
      mask help: Bus block.
      mask init:
      | fm_inout
      settings: AttributesFormatString="|V| =  0.9846 p.u.\\n<V  = -0.1289 rad"
      mask CallbackString: ||||fm_block|
      mask Display: plot([0 1 1 0 0],[0 0 1 1 0])
  Planta Centro 400kV : PMComponent  Tag=PSATblock  Description=Connection  PhysicalDomain=psatdomain  LeftPortType=p1  RightPortType=p1  LConnTagsString=__newl0|__newl1|__newl2  RConnTagsString=__newr0|__newr1|__newr2|__newr3  mask(Bus){in=3, out=4, p2q=400, p3_4q=[1.05    -0.41469], p5q=1, p6q=1}
      mask prompts: in "Number of inputs:"; out "Number of outputs:"; p2q "Voltage Rating [kV]"; p3_4q "Voltage initial guess [p.u.  rad]"; p5q "Area number"; p6q "Region number"
      mask help: Bus block.
      mask init:
      | fm_inout
      settings: AttributesFormatString="|V| =  1.04   p.u.\\n<V  = -0.0886 rad"
      mask CallbackString: ||||fm_block|
      mask Display: plot([0 1 1 0 0],[0 0 1 1 0])
  Planta Paez 115kV : PMComponent  Tag=PSATblock  Description=Connection  PhysicalDomain=psatdomain  LeftPortType=p1  RightPortType=p1  LConnTagsString=__newl0|__newl1|__newl2|__newl3|__newl4  RConnTagsString=__newr0|__newr1|__newr2|__newr3  mask(Bus){in=5, out=4, p2q=115, p3_4q=[0.98444    -0.26004], p5q=1, p6q=1}
      mask prompts: in "Number of inputs:"; out "Number of outputs:"; p2q "Voltage Rating [kV]"; p3_4q "Voltage initial guess [p.u.  rad]"; p5q "Area number"; p6q "Region number"
      mask help: Bus block.
      mask init:
      | fm_inout
      settings: AttributesFormatString="|V| =  1.04   p.u.\\n<V  =  0.1292 rad"
      mask CallbackString: ||||fm_block|
      mask Display: plot([0 1 1 0 0],[0 0 1 1 0])
  Planta Paez 230kV : PMComponent  Tag=PSATblock  Description=Connection  PhysicalDomain=psatdomain  LeftPortType=p1  RightPortType=p1  LConnTagsString=__newl0|__newl1|__newl2  RConnTagsString=__newr0|__newr1|__newr2  mask(Bus){in=3, out=3, p2q=230, p3_4q=[1.07    -0.62878], p5q=1, p6q=1}
      mask prompts: in "Number of inputs:"; out "Number of outputs:"; p2q "Voltage Rating [kV]"; p3_4q "Voltage initial guess [p.u.  rad]"; p5q "Area number"; p6q "Region number"
      mask help: Bus block.
      mask init:
      | fm_inout
      settings: AttributesFormatString="|V| =  1.04   p.u.\\n<V  =  0.1523 rad"
      mask CallbackString: ||||fm_block|
      mask Display: plot([0 1 1 0 0],[0 0 1 1 0])
  Planta Tachira : PMComponent  Tag=PSATblock  Description=Connection  PhysicalDomain=psatdomain  LeftPortType=p1  RightPortType=p1  LConnTagsString=__newl0|__newl1|__newl2|__newl3  RConnTagsString=__newr0|__newr1|__newr2|__newr3  mask(Bus){in=4, out=4, p2q=115, p3_4q=[0.98444    -0.26004], p5q=1, p6q=1}
      mask prompts: in "Number of inputs:"; out "Number of outputs:"; p2q "Voltage Rating [kV]"; p3_4q "Voltage initial guess [p.u.  rad]"; p5q "Area number"; p6q "Region number"
      mask help: Bus block.
      mask init:
      | fm_inout
      settings: AttributesFormatString="|V| =  1.02   p.u.\\n<V  =  0.4800 rad"
      mask CallbackString: ||||fm_block|
      mask Display: plot([0 1 1 0 0],[0 0 1 1 0])
  Punto Fijo I : PMComponent  Tag=PSATblock  Description=Connection  PhysicalDomain=psatdomain  LeftPortType=p1  RightPortType=p1  LConnTagsString=__newl0|__newl1  RConnTagsString=__newr0|__newr1  mask(Bus){in=2, out=2, p2q=115, p3_4q=[1.02    0.054618], p5q=1, p6q=1}
      mask prompts: in "Number of inputs:"; out "Number of outputs:"; p2q "Voltage Rating [kV]"; p3_4q "Voltage initial guess [p.u.  rad]"; p5q "Area number"; p6q "Region number"
      mask help: Bus block.
      mask init:
      | fm_inout
      settings: AttributesFormatString="|V| =  1.04   p.u.\\n<V  =  0.7803 rad"
      mask CallbackString: ||||fm_block|
      mask Display: plot([0 1 1 0 0],[0 0 1 1 0])
  Punto Fijo II : PMComponent  Tag=PSATblock  Description=Connection  PhysicalDomain=psatdomain  LeftPortType=p1  RightPortType=p1  LConnTagsString=__newl0|__newl1  RConnTagsString=__newr0|__newr1|__newr2  mask(Bus){in=2, out=3, p2q=115, p3_4q=[0.99383    0.019735], p5q=1, p6q=1}
      mask prompts: in "Number of inputs:"; out "Number of outputs:"; p2q "Voltage Rating [kV]"; p3_4q "Voltage initial guess [p.u.  rad]"; p5q "Area number"; p6q "Region number"
      mask help: Bus block.
      mask init:
      | fm_inout
      settings: AttributesFormatString="|V| =  1.0203 p.u.\\n<V  =  0.7450 rad"
      mask CallbackString: ||||fm_block|
      mask Display: plot([0 1 1 0 0],[0 0 1 1 0])
  Puricaure : PMComponent  Tag=PSATblock  Description=Connection  PhysicalDomain=psatdomain  LeftPortType=p1  RightPortType=p1  LConnTagsString=__newl0  RConnTagsString=__newr0  mask(Bus){in=1, out=1, p2q=115, p3_4q=[1.0023    -0.25717], p5q=1, p6q=1}
      mask prompts: in "Number of inputs:"; out "Number of outputs:"; p2q "Voltage Rating [kV]"; p3_4q "Voltage initial guess [p.u.  rad]"; p5q "Area number"; p6q "Region number"
      mask help: Bus block.
      mask init:
      | fm_inout
      settings: AttributesFormatString="|V| =  1.0107 p.u.\\n<V  =  0.0245 rad"
      mask CallbackString: ||||fm_block|
      mask Display: plot([0 1 1 0 0],[0 0 1 1 0])
  Ramon Laguna 138kV : PMComponent  Tag=PSATblock  Description=Connection  PhysicalDomain=psatdomain  LeftPortType=p1  RightPortType=p1  LConnTagsString=__newl0|__newl1|__newl2|__newl3|__newl4  RConnTagsString=__newr0|__newr1  mask(Bus){in=5, out=2, p2q=138, p3_4q=[1.07    -0.91379], p5q=1, p6q=1}
      mask prompts: in "Number of inputs:"; out "Number of outputs:"; p2q "Voltage Rating [kV]"; p3_4q "Voltage initial guess [p.u.  rad]"; p5q "Area number"; p6q "Region number"
      mask help: Bus block.
      mask init:
      | fm_inout
      settings: AttributesFormatString="|V| =  1.04   p.u.\\n<V  =  0.0297 rad"
      mask CallbackString: ||||fm_block|
      mask Display: plot([0 1 1 0 0],[0 0 1 1 0])
  Rio Chico II : PMComponent  Tag=PSATblock  Description=Connection  PhysicalDomain=psatdomain  LeftPortType=p1  RightPortType=p1  LConnTagsString=__newl0|__newl1  RConnTagsString=__newr0  mask(Bus){in=2, out=1, p2q=230, p3_4q=[0.92904    -0.47497], p5q=1, p6q=1}
      mask prompts: in "Number of inputs:"; out "Number of outputs:"; p2q "Voltage Rating [kV]"; p3_4q "Voltage initial guess [p.u.  rad]"; p5q "Area number"; p6q "Region number"
      mask help: Bus block.
      mask init:
      | fm_inout
      settings: AttributesFormatString="|V| =  0.9835 p.u.\\n<V  = -0.1821 rad"
      mask CallbackString: ||||fm_block|
      mask Display: plot([0 1 1 0 0],[0 0 1 1 0])
  SC1 : PMComponent  Tag=PSATblock  Description=Power Flow  PhysicalDomain=psatdomain  LeftPortType=p1  RightPortType=p1  RConnTagsString=__newr0  mask(PV){p2_3q=[100  765], p5q=1.04, p6_7q=[2.8  -3], p8_9q=[1.1  0.9], p10q=1, p11q=on}
      mask prompts: p2_3q "Power and Voltage Ratings [MVA, kV]"; p5q "Voltage Magnitude [p.u.]"; p6_7q "Qmax and Qmin [p.u.  p.u.]"; p8_9q "Vmax and Vmin [p.u.  p.u.]"; p10q "Loss Participation Coefficient"; p11q "Connected"
      mask help:
      | This block defines a static synchronous compensator:
      | P = 0
      | V = Vdes
      mask init:
      | [x,y] = fm_draw('circle');
      | [xc,yc] = fm_draw('C');
      mask CallbackString: |||||fm_block
      mask Display:
      | plot(x,y,[-0.25 -0.25],[-0.25 0.25])
      | color('blue')
      | plot(0.5*xc-0.25,yc)
  SC3 : PMComponent  Tag=PSATblock  Description=Power Flow  PhysicalDomain=psatdomain  LeftPortType=p1  RightPortType=p1  RConnTagsString=__newr0  mask(PV){p2_3q=[100  765], p5q=1.04, p6_7q=[2.8  -3], p8_9q=[1.1  0.9], p10q=1, p11q=on}
      mask prompts: p2_3q "Power and Voltage Ratings [MVA, kV]"; p5q "Voltage Magnitude [p.u.]"; p6_7q "Qmax and Qmin [p.u.  p.u.]"; p8_9q "Vmax and Vmin [p.u.  p.u.]"; p10q "Loss Participation Coefficient"; p11q "Connected"
      mask help:
      | This block defines a static synchronous compensator:
      | P = 0
      | V = Vdes
      mask init:
      | [x,y] = fm_draw('circle');
      | [xc,yc] = fm_draw('C');
      mask CallbackString: |||||fm_block
      mask Display:
      | plot(x,y,[-0.25 -0.25],[-0.25 0.25])
      | color('blue')
      | plot(0.5*xc-0.25,yc)
  San Agaton 230kV : PMComponent  Tag=PSATblock  Description=Connection  PhysicalDomain=psatdomain  LeftPortType=p1  RightPortType=p1  LConnTagsString=__newl0|__newl1  RConnTagsString=__newr0|__newr1  mask(Bus){in=2, out=2, p2q=230, p3_4q=[1.07    -0.64372], p5q=1, p6q=1}
      mask prompts: in "Number of inputs:"; out "Number of outputs:"; p2q "Voltage Rating [kV]"; p3_4q "Voltage initial guess [p.u.  rad]"; p5q "Area number"; p6q "Region number"
      mask help: Bus block.
      mask init:
      | fm_inout
      settings: AttributesFormatString="|V| =  1.02   p.u.\\n<V  =  0.5689 rad"
      mask CallbackString: ||||fm_block|
      mask Display: plot([0 1 1 0 0],[0 0 1 1 0])
  San Antonio : PMComponent  Tag=PSATblock  Description=Connection  PhysicalDomain=psatdomain  LeftPortType=p1  RightPortType=p1  LConnTagsString=__newl0|__newl1  RConnTagsString=__newr0|__newr1  mask(Bus){in=2, out=2, p2q=115, p3_4q=[1.0023    -0.25717], p5q=1, p6q=1}
      mask prompts: in "Number of inputs:"; out "Number of outputs:"; p2q "Voltage Rating [kV]"; p3_4q "Voltage initial guess [p.u.  rad]"; p5q "Area number"; p6q "Region number"
      mask help: Bus block.
      mask init:
      | fm_inout
      settings: AttributesFormatString="|V| =  1.0181 p.u.\\n<V  =  0.4567 rad"
      mask CallbackString: ||||fm_block|
      mask Display: plot([0 1 1 0 0],[0 0 1 1 0])
  San Carlos del Zulia : PMComponent  Tag=PSATblock  Description=Connection  PhysicalDomain=psatdomain  LeftPortType=p1  RightPortType=p1  LConnTagsString=__newl0|__newl1  RConnTagsString=__newr0  mask(Bus){in=2, out=1, p2q=115, p3_4q=[1.0023    -0.25717], p5q=1, p6q=1}
      mask prompts: in "Number of inputs:"; out "Number of outputs:"; p2q "Voltage Rating [kV]"; p3_4q "Voltage initial guess [p.u.  rad]"; p5q "Area number"; p6q "Region number"
      mask help: Bus block.
      mask init:
      | fm_inout
      settings: AttributesFormatString="|V| =  1.04   p.u.\\n<V  =  0.4909 rad"
      mask CallbackString: ||||fm_block|
      mask Display: plot([0 1 1 0 0],[0 0 1 1 0])
  San Cristobal I : PMComponent  Tag=PSATblock  Description=Connection  PhysicalDomain=psatdomain  LeftPortType=p1  RightPortType=p1  LConnTagsString=__newl0|__newl1  RConnTagsString=__newr0|__newr1  mask(Bus){in=2, out=2, p2q=115, p3_4q=[1.0023    -0.25717], p5q=1, p6q=1}
      mask prompts: in "Number of inputs:"; out "Number of outputs:"; p2q "Voltage Rating [kV]"; p3_4q "Voltage initial guess [p.u.  rad]"; p5q "Area number"; p6q "Region number"
      mask help: Bus block.
      mask init:
      | fm_inout
      settings: AttributesFormatString="|V| =  1.0137 p.u.\\n<V  =  0.4515 rad"
      mask CallbackString: ||||fm_block|
      mask Display: plot([0 1 1 0 0],[0 0 1 1 0])
  San Cristobal II : PMComponent  Tag=PSATblock  Description=Connection  PhysicalDomain=psatdomain  LeftPortType=p1  RightPortType=p1  LConnTagsString=__newl0  RConnTagsString=__newr0|__newr1  mask(Bus){in=1, out=2, p2q=115, p3_4q=[1.0023    -0.25717], p5q=1, p6q=1}
      mask prompts: in "Number of inputs:"; out "Number of outputs:"; p2q "Voltage Rating [kV]"; p3_4q "Voltage initial guess [p.u.  rad]"; p5q "Area number"; p6q "Region number"
      mask help: Bus block.
      mask init:
      | fm_inout
      settings: AttributesFormatString="|V| =  1.0144 p.u.\\n<V  =  0.4624 rad"
      mask CallbackString: ||||fm_block|
      mask Display: plot([0 1 1 0 0],[0 0 1 1 0])
  San Diego 230kV : PMComponent  Tag=PSATblock  Description=Connection  PhysicalDomain=psatdomain  LeftPortType=p1  RightPortType=p1  LConnTagsString=__newl0|__newl1|__newl2|__newl3  RConnTagsString=__newr0|__newr1|__newr2  mask(Bus){in=4, out=3, p2q=230, p3_4q=[0.94718     -0.5857], p5q=1, p6q=1}
      mask prompts: in "Number of inputs:"; out "Number of outputs:"; p2q "Voltage Rating [kV]"; p3_4q "Voltage initial guess [p.u.  rad]"; p5q "Area number"; p6q "Region number"
      mask help: Bus block.
      mask init:
      | fm_inout
      settings: AttributesFormatString="|V| =  1.04   p.u.\\n<V  = -0.2814 rad"
      mask CallbackString: ||||fm_block|
      mask Display: plot([0 1 1 0 0],[0 0 1 1 0])
  San Fernando II 230kV : PMComponent  Tag=PSATblock  Description=Connection  PhysicalDomain=psatdomain  LeftPortType=p1  RightPortType=p1  LConnTagsString=__newl0|__newl1  RConnTagsString=__newr0  mask(Bus){in=2, out=1, p2q=230, p3_4q=[1.0021    -0.55915], p5q=1, p6q=1}
      mask prompts: in "Number of inputs:"; out "Number of outputs:"; p2q "Voltage Rating [kV]"; p3_4q "Voltage initial guess [p.u.  rad]"; p5q "Area number"; p6q "Region number"
      mask help: Bus block.
      mask init:
      | fm_inout
      settings: AttributesFormatString="|V| =  1.0339 p.u.\\n<V  = -0.1713 rad"
      mask CallbackString: ||||fm_block|
      mask Display: plot([0 1 1 0 0],[0 0 1 1 0])
  San Geronimo 400kV : PMComponent  Tag=PSATblock  Description=Connection  PhysicalDomain=psatdomain  LeftPortType=p1  RightPortType=p1  LConnTagsString=__newl0|__newl1|__newl2|__newl3|__newl4  RConnTagsString=__newr0|__newr1|__newr2  mask(Bus){in=5, out=3, p2q=400, p3_4q=[1.0293    -0.26664], p5q=1, p6q=1}
      mask prompts: in "Number of inputs:"; out "Number of outputs:"; p2q "Voltage Rating [kV]"; p3_4q "Voltage initial guess [p.u.  rad]"; p5q "Area number"; p6q "Region number"
      mask help: Bus block.
      mask init:
      | fm_inout
      settings: AttributesFormatString="|V| =  1.0412 p.u.\\n<V  = -0.0900 rad"
      mask CallbackString: ||||fm_block|
      mask Display: plot([0 1 1 0 0],[0 0 1 1 0])
  San Geronimo 765kV : PMComponent  Tag=PSATblock  Description=Connection  PhysicalDomain=psatdomain  LeftPortType=p1  RightPortType=p1  LConnTagsString=__newl0|__newl1|__newl2|__newl3|__newl4  RConnTagsString=__newr0|__newr1|__newr2|__newr3|__newr4|__newr5  mask(Bus){in=5, out=6, p2q=765, p3_4q=[1.05     -0.2544], p5q=1, p6q=1}
      mask prompts: in "Number of inputs:"; out "Number of outputs:"; p2q "Voltage Rating [kV]"; p3_4q "Voltage initial guess [p.u.  rad]"; p5q "Area number"; p6q "Region number"
      mask help: Bus block.
      mask init:
      | fm_inout
      settings: AttributesFormatString="|V| =  1.04   p.u.\\n<V  = -0.0906 rad"
      mask CallbackString: ||||fm_block|
      mask Display: plot([0 1 1 0 0],[0 0 1 1 0])
  San Lorenzo : PMComponent  Tag=PSATblock  Description=Connection  PhysicalDomain=psatdomain  LeftPortType=p1  RightPortType=p1  LConnTagsString=__newl0|__newl1|__newl2|__newl3  RConnTagsString=__newr0|__newr1  mask(Bus){in=4, out=2, p2q=115, p3_4q=[0.98444    -0.26004], p5q=1, p6q=1}
      mask prompts: in "Number of inputs:"; out "Number of outputs:"; p2q "Voltage Rating [kV]"; p3_4q "Voltage initial guess [p.u.  rad]"; p5q "Area number"; p6q "Region number"
      mask help: Bus block.
      mask init:
      | fm_inout
      settings: AttributesFormatString="|V| =  1.02   p.u.\\n<V  =  0.0377 rad"
      mask CallbackString: ||||fm_block|
      mask Display: plot([0 1 1 0 0],[0 0 1 1 0])
  San Mateo 230kV : PMComponent  Tag=PSATblock  Description=Connection  PhysicalDomain=psatdomain  LeftPortType=p1  RightPortType=p1  LConnTagsString=__newl0  RConnTagsString=__newr0|__newr1  mask(Bus){in=1, out=2, p2q=230, p3_4q=[1.0593    -0.69162], p5q=1, p6q=1}
      mask prompts: in "Number of inputs:"; out "Number of outputs:"; p2q "Voltage Rating [kV]"; p3_4q "Voltage initial guess [p.u.  rad]"; p5q "Area number"; p6q "Region number"
      mask help: Bus block.
      mask init:
      | fm_inout
      settings: AttributesFormatString="|V| =  1.064  p.u.\\n<V  =  0.5269 rad"
      mask CallbackString: ||||fm_block|
      mask Display: plot([0 1 1 0 0],[0 0 1 1 0])
  Santa Elena : PMComponent  Tag=PSATblock  Description=Connection  PhysicalDomain=psatdomain  LeftPortType=p1  RightPortType=p1  LConnTagsString=__newl0|__newl1  RConnTagsString=__newr0  mask(Bus){in=2, out=1, p2q=230, p3_4q=[1.0158    -0.30624], p5q=1, p6q=1}
      mask prompts: in "Number of inputs:"; out "Number of outputs:"; p2q "Voltage Rating [kV]"; p3_4q "Voltage initial guess [p.u.  rad]"; p5q "Area number"; p6q "Region number"
      mask help: Bus block.
      mask init:
      | fm_inout
      settings: AttributesFormatString="|V| =  0.9914 p.u.\\n<V  = -0.2852 rad"
      mask CallbackString: ||||fm_block|
      mask Display: plot([0 1 1 0 0],[0 0 1 1 0])
  Santa Teresa 230kV : PMComponent  Tag=PSATblock  Description=Connection  PhysicalDomain=psatdomain  LeftPortType=p1  RightPortType=p1  LConnTagsString=__newl0|__newl1|__newl2|__newl3|__newl4|__newl5  RConnTagsString=__newr0|__newr1|__newr2|__newr3|__newr4  mask(Bus){in=6, out=5, p2q=230, p3_4q=[0.93698    -0.47554], p5q=1, p6q=1}
      mask prompts: in "Number of inputs:"; out "Number of outputs:"; p2q "Voltage Rating [kV]"; p3_4q "Voltage initial guess [p.u.  rad]"; p5q "Area number"; p6q "Region number"
      mask help: Bus block.
      mask init:
      | fm_inout
      settings: AttributesFormatString="|V| =  1.0062 p.u.\\n<V  = -0.1750 rad"
      mask CallbackString: ||||fm_block|
      mask Display: plot([0 1 1 0 0],[0 0 1 1 0])
  Santa Teresa 400kV : PMComponent  Tag=PSATblock  Description=Connection  PhysicalDomain=psatdomain  LeftPortType=p1  RightPortType=p1  LConnTagsString=__newl0|__newl1  RConnTagsString=__newr0|__newr1|__newr2|__newr3  mask(Bus){in=2, out=4, p2q=400, p3_4q=[0.90882     -0.3702], p5q=1, p6q=1}
      mask prompts: in "Number of inputs:"; out "Number of outputs:"; p2q "Voltage Rating [kV]"; p3_4q "Voltage initial guess [p.u.  rad]"; p5q "Area number"; p6q "Region number"
      mask help: Bus block.
      mask init:
      | fm_inout
      settings: AttributesFormatString="|V| =  1.017  p.u.\\n<V  = -0.1567 rad"
      mask CallbackString: ||||fm_block|
      mask Display: plot([0 1 1 0 0],[0 0 1 1 0])
  Shunt1 : PMComponent  Tag=PSATblock  Description=Power Flow  PhysicalDomain=psatdomain  LeftPortType=p1  RightPortType=p1  LConnTagsString=__newl0  mask(Shunt){p2_3_4q=[100  115  60], p6q=0.12, p7q=on}
      mask prompts: p2_3_4q "Power, Voltage and Frequency Ratings [MVA, kV, Hz]"; p6q "Susceptance B [p.u.]"; p7q "Connected"
      mask help:
      | This block defines a static condenser:
      |
      | Q = B * V^2
      |
      | (Negative values of B define an inductive load).
      mask init:
      | fm_block
      mask CallbackString: ||fm_block
      mask Display: plot(-[0 60 60 55 53 55 60 60 55 53]/150,[0 0 8 16 25 16 8 -8 -16 -25]/50,-[80 80 80 150]/150,[25 -25 0 0]/50,[0 0],[-0.4 0.4],[0.075 0.075],[-0.25 0.25],[0.15 0.15],[-0.1 0.1])
  Shunt10 : PMComponent  Tag=PSATblock  Description=Power Flow  PhysicalDomain=psatdomain  LeftPortType=p1  RightPortType=p1  LConnTagsString=__newl0  mask(Shunt){p2_3_4q=[100  115  60], p6q=0.12, p7q=on}
      mask prompts: p2_3_4q "Power, Voltage and Frequency Ratings [MVA, kV, Hz]"; p6q "Susceptance B [p.u.]"; p7q "Connected"
      mask help:
      | This block defines a static condenser:
      |
      | Q = B * V^2
      |
      | (Negative values of B define an inductive load).
      mask init:
      | fm_block
      mask CallbackString: ||fm_block
      mask Display: plot(-[0 60 60 55 53 55 60 60 55 53]/150,[0 0 8 16 25 16 8 -8 -16 -25]/50,-[80 80 80 150]/150,[25 -25 0 0]/50,[0 0],[-0.4 0.4],[0.075 0.075],[-0.25 0.25],[0.15 0.15],[-0.1 0.1])
  Shunt11 : PMComponent  Tag=PSATblock  Description=Power Flow  PhysicalDomain=psatdomain  LeftPortType=p1  RightPortType=p1  LConnTagsString=__newl0  mask(Shunt){p2_3_4q=[100  115  60], p6q=0.12, p7q=on}
      mask prompts: p2_3_4q "Power, Voltage and Frequency Ratings [MVA, kV, Hz]"; p6q "Susceptance B [p.u.]"; p7q "Connected"
      mask help:
      | This block defines a static condenser:
      |
      | Q = B * V^2
      |
      | (Negative values of B define an inductive load).
      mask init:
      | fm_block
      mask CallbackString: ||fm_block
      mask Display: plot(-[0 60 60 55 53 55 60 60 55 53]/150,[0 0 8 16 25 16 8 -8 -16 -25]/50,-[80 80 80 150]/150,[25 -25 0 0]/50,[0 0],[-0.4 0.4],[0.075 0.075],[-0.25 0.25],[0.15 0.15],[-0.1 0.1])
  Shunt12 : PMComponent  Tag=PSATblock  Description=Power Flow  PhysicalDomain=psatdomain  LeftPortType=p1  RightPortType=p1  LConnTagsString=__newl0  mask(Shunt){p2_3_4q=[100  115  60], p6q=0.12, p7q=on}
      mask prompts: p2_3_4q "Power, Voltage and Frequency Ratings [MVA, kV, Hz]"; p6q "Susceptance B [p.u.]"; p7q "Connected"
      mask help:
      | This block defines a static condenser:
      |
      | Q = B * V^2
      |
      | (Negative values of B define an inductive load).
      mask init:
      | fm_block
      mask CallbackString: ||fm_block
      mask Display: plot(-[0 60 60 55 53 55 60 60 55 53]/150,[0 0 8 16 25 16 8 -8 -16 -25]/50,-[80 80 80 150]/150,[25 -25 0 0]/50,[0 0],[-0.4 0.4],[0.075 0.075],[-0.25 0.25],[0.15 0.15],[-0.1 0.1])
  Shunt13 : PMComponent  Tag=PSATblock  Description=Power Flow  PhysicalDomain=psatdomain  LeftPortType=p1  RightPortType=p1  LConnTagsString=__newl0  mask(Shunt){p2_3_4q=[100  115  60], p6q=0.03, p7q=on}
      mask prompts: p2_3_4q "Power, Voltage and Frequency Ratings [MVA, kV, Hz]"; p6q "Susceptance B [p.u.]"; p7q "Connected"
      mask help:
      | This block defines a static condenser:
      |
      | Q = B * V^2
      |
      | (Negative values of B define an inductive load).
      mask init:
      | fm_block
      mask CallbackString: ||fm_block
      mask Display: plot(-[0 60 60 55 53 55 60 60 55 53]/150,[0 0 8 16 25 16 8 -8 -16 -25]/50,-[80 80 80 150]/150,[25 -25 0 0]/50,[0 0],[-0.4 0.4],[0.075 0.075],[-0.25 0.25],[0.15 0.15],[-0.1 0.1])
  Shunt14 : PMComponent  Tag=PSATblock  Description=Power Flow  PhysicalDomain=psatdomain  LeftPortType=p1  RightPortType=p1  LConnTagsString=__newl0  mask(Shunt){p2_3_4q=[100  115  60], p6q=0.09, p7q=on}
      mask prompts: p2_3_4q "Power, Voltage and Frequency Ratings [MVA, kV, Hz]"; p6q "Susceptance B [p.u.]"; p7q "Connected"
      mask help:
      | This block defines a static condenser:
      |
      | Q = B * V^2
      |
      | (Negative values of B define an inductive load).
      mask init:
      | fm_block
      mask CallbackString: ||fm_block
      mask Display: plot(-[0 60 60 55 53 55 60 60 55 53]/150,[0 0 8 16 25 16 8 -8 -16 -25]/50,-[80 80 80 150]/150,[25 -25 0 0]/50,[0 0],[-0.4 0.4],[0.075 0.075],[-0.25 0.25],[0.15 0.15],[-0.1 0.1])
  Shunt15 : PMComponent  Tag=PSATblock  Description=Power Flow  PhysicalDomain=psatdomain  LeftPortType=p1  RightPortType=p1  LConnTagsString=__newl0  mask(Shunt){p2_3_4q=[100  115  60], p6q=0.015, p7q=on}
      mask prompts: p2_3_4q "Power, Voltage and Frequency Ratings [MVA, kV, Hz]"; p6q "Susceptance B [p.u.]"; p7q "Connected"
      mask help:
      | This block defines a static condenser:
      |
      | Q = B * V^2
      |
      | (Negative values of B define an inductive load).
      mask init:
      | fm_block
      mask CallbackString: ||fm_block
      mask Display: plot(-[0 60 60 55 53 55 60 60 55 53]/150,[0 0 8 16 25 16 8 -8 -16 -25]/50,-[80 80 80 150]/150,[25 -25 0 0]/50,[0 0],[-0.4 0.4],[0.075 0.075],[-0.25 0.25],[0.15 0.15],[-0.1 0.1])
  Shunt16 : PMComponent  Tag=PSATblock  Description=Power Flow  PhysicalDomain=psatdomain  LeftPortType=p1  RightPortType=p1  LConnTagsString=__newl0  mask(Shunt){p2_3_4q=[100  115  60], p6q=0.06, p7q=on}
      mask prompts: p2_3_4q "Power, Voltage and Frequency Ratings [MVA, kV, Hz]"; p6q "Susceptance B [p.u.]"; p7q "Connected"
      mask help:
      | This block defines a static condenser:
      |
      | Q = B * V^2
      |
      | (Negative values of B define an inductive load).
      mask init:
      | fm_block
      mask CallbackString: ||fm_block
      mask Display: plot(-[0 60 60 55 53 55 60 60 55 53]/150,[0 0 8 16 25 16 8 -8 -16 -25]/50,-[80 80 80 150]/150,[25 -25 0 0]/50,[0 0],[-0.4 0.4],[0.075 0.075],[-0.25 0.25],[0.15 0.15],[-0.1 0.1])
  Shunt17 : PMComponent  Tag=PSATblock  Description=Power Flow  PhysicalDomain=psatdomain  LeftPortType=p1  RightPortType=p1  LConnTagsString=__newl0  mask(Shunt){p2_3_4q=[100  115  60], p6q=0.06, p7q=on}
      mask prompts: p2_3_4q "Power, Voltage and Frequency Ratings [MVA, kV, Hz]"; p6q "Susceptance B [p.u.]"; p7q "Connected"
      mask help:
      | This block defines a static condenser:
      |
      | Q = B * V^2
      |
      | (Negative values of B define an inductive load).
      mask init:
      | fm_block
      mask CallbackString: ||fm_block
      mask Display: plot(-[0 60 60 55 53 55 60 60 55 53]/150,[0 0 8 16 25 16 8 -8 -16 -25]/50,-[80 80 80 150]/150,[25 -25 0 0]/50,[0 0],[-0.4 0.4],[0.075 0.075],[-0.25 0.25],[0.15 0.15],[-0.1 0.1])
  Shunt18 : PMComponent  Tag=PSATblock  Description=Power Flow  PhysicalDomain=psatdomain  LeftPortType=p1  RightPortType=p1  LConnTagsString=__newl0  mask(Shunt){p2_3_4q=[100  115  60], p6q=0.24, p7q=on}
      mask prompts: p2_3_4q "Power, Voltage and Frequency Ratings [MVA, kV, Hz]"; p6q "Susceptance B [p.u.]"; p7q "Connected"
      mask help:
      | This block defines a static condenser:
      |
      | Q = B * V^2
      |
      | (Negative values of B define an inductive load).
      mask init:
      | fm_block
      mask CallbackString: ||fm_block
      mask Display: plot(-[0 60 60 55 53 55 60 60 55 53]/150,[0 0 8 16 25 16 8 -8 -16 -25]/50,-[80 80 80 150]/150,[25 -25 0 0]/50,[0 0],[-0.4 0.4],[0.075 0.075],[-0.25 0.25],[0.15 0.15],[-0.1 0.1])
  Shunt19 : PMComponent  Tag=PSATblock  Description=Power Flow  PhysicalDomain=psatdomain  LeftPortType=p1  RightPortType=p1  LConnTagsString=__newl0  mask(Shunt){p2_3_4q=[100  115  60], p6q=0.12, p7q=on}
      mask prompts: p2_3_4q "Power, Voltage and Frequency Ratings [MVA, kV, Hz]"; p6q "Susceptance B [p.u.]"; p7q "Connected"
      mask help:
      | This block defines a static condenser:
      |
      | Q = B * V^2
      |
      | (Negative values of B define an inductive load).
      mask init:
      | fm_block
      mask CallbackString: ||fm_block
      mask Display: plot(-[0 60 60 55 53 55 60 60 55 53]/150,[0 0 8 16 25 16 8 -8 -16 -25]/50,-[80 80 80 150]/150,[25 -25 0 0]/50,[0 0],[-0.4 0.4],[0.075 0.075],[-0.25 0.25],[0.15 0.15],[-0.1 0.1])
  Shunt2 : PMComponent  Tag=PSATblock  Description=Power Flow  PhysicalDomain=psatdomain  LeftPortType=p1  RightPortType=p1  LConnTagsString=__newl0  mask(Shunt){p2_3_4q=[100  230  60], p6q=1.08, p7q=on}
      mask prompts: p2_3_4q "Power, Voltage and Frequency Ratings [MVA, kV, Hz]"; p6q "Susceptance B [p.u.]"; p7q "Connected"
      mask help:
      | This block defines a static condenser:
      |
      | Q = B * V^2
      |
      | (Negative values of B define an inductive load).
      mask init:
      | fm_block
      mask CallbackString: ||fm_block
      mask Display: plot(-[0 60 60 55 53 55 60 60 55 53]/150,[0 0 8 16 25 16 8 -8 -16 -25]/50,-[80 80 80 150]/150,[25 -25 0 0]/50,[0 0],[-0.4 0.4],[0.075 0.075],[-0.25 0.25],[0.15 0.15],[-0.1 0.1])
  Shunt3 : PMComponent  Tag=PSATblock  Description=Power Flow  PhysicalDomain=psatdomain  LeftPortType=p1  RightPortType=p1  LConnTagsString=__newl0  mask(Shunt){p2_3_4q=[100  115  60], p6q=0.000907372, p7q=off}
      mask prompts: p2_3_4q "Power, Voltage and Frequency Ratings [MVA, kV, Hz]"; p6q "Susceptance B [p.u.]"; p7q "Connected"
      mask help:
      | This block defines a static condenser:
      |
      | Q = B * V^2
      |
      | (Negative values of B define an inductive load).
      mask init:
      | fm_block
      mask CallbackString: ||fm_block
      mask Display: plot(-[0 60 60 55 53 55 60 60 55 53]/150,[0 0 8 16 25 16 8 -8 -16 -25]/50,-[80 80 80 150]/150,[25 -25 0 0]/50,[0 0],[-0.4 0.4],[0.075 0.075],[-0.25 0.25],[0.15 0.15],[-0.1 0.1])
  Shunt4 : PMComponent  Tag=PSATblock  Description=Power Flow  PhysicalDomain=psatdomain  LeftPortType=p1  RightPortType=p1  LConnTagsString=__newl0  mask(Shunt){p2_3_4q=[100  230  60], p6q=0.8, p7q=on}
      mask prompts: p2_3_4q "Power, Voltage and Frequency Ratings [MVA, kV, Hz]"; p6q "Susceptance B [p.u.]"; p7q "Connected"
      mask help:
      | This block defines a static condenser:
      |
      | Q = B * V^2
      |
      | (Negative values of B define an inductive load).
      mask init:
      | fm_block
      mask CallbackString: ||fm_block
      mask Display: plot(-[0 60 60 55 53 55 60 60 55 53]/150,[0 0 8 16 25 16 8 -8 -16 -25]/50,-[80 80 80 150]/150,[25 -25 0 0]/50,[0 0],[-0.4 0.4],[0.075 0.075],[-0.25 0.25],[0.15 0.15],[-0.1 0.1])
  Shunt7 : PMComponent  Tag=PSATblock  Description=Power Flow  PhysicalDomain=psatdomain  LeftPortType=p1  RightPortType=p1  LConnTagsString=__newl0  mask(Shunt){p2_3_4q=[100  115  60], p6q=0.12, p7q=on}
      mask prompts: p2_3_4q "Power, Voltage and Frequency Ratings [MVA, kV, Hz]"; p6q "Susceptance B [p.u.]"; p7q "Connected"
      mask help:
      | This block defines a static condenser:
      |
      | Q = B * V^2
      |
      | (Negative values of B define an inductive load).
      mask init:
      | fm_block
      mask CallbackString: ||fm_block
      mask Display: plot(-[0 60 60 55 53 55 60 60 55 53]/150,[0 0 8 16 25 16 8 -8 -16 -25]/50,-[80 80 80 150]/150,[25 -25 0 0]/50,[0 0],[-0.4 0.4],[0.075 0.075],[-0.25 0.25],[0.15 0.15],[-0.1 0.1])
  Shunt8 : PMComponent  Tag=PSATblock  Description=Power Flow  PhysicalDomain=psatdomain  LeftPortType=p1  RightPortType=p1  LConnTagsString=__newl0  mask(Shunt){p2_3_4q=[100  115  60], p6q=0.12, p7q=on}
      mask prompts: p2_3_4q "Power, Voltage and Frequency Ratings [MVA, kV, Hz]"; p6q "Susceptance B [p.u.]"; p7q "Connected"
      mask help:
      | This block defines a static condenser:
      |
      | Q = B * V^2
      |
      | (Negative values of B define an inductive load).
      mask init:
      | fm_block
      mask CallbackString: ||fm_block
      mask Display: plot(-[0 60 60 55 53 55 60 60 55 53]/150,[0 0 8 16 25 16 8 -8 -16 -25]/50,-[80 80 80 150]/150,[25 -25 0 0]/50,[0 0],[-0.4 0.4],[0.075 0.075],[-0.25 0.25],[0.15 0.15],[-0.1 0.1])
  Shunt9 : PMComponent  Tag=PSATblock  Description=Power Flow  PhysicalDomain=psatdomain  LeftPortType=p1  RightPortType=p1  LConnTagsString=__newl0  mask(Shunt){p2_3_4q=[100  115  60], p6q=0.12, p7q=on}
      mask prompts: p2_3_4q "Power, Voltage and Frequency Ratings [MVA, kV, Hz]"; p6q "Susceptance B [p.u.]"; p7q "Connected"
      mask help:
      | This block defines a static condenser:
      |
      | Q = B * V^2
      |
      | (Negative values of B define an inductive load).
      mask init:
      | fm_block
      mask CallbackString: ||fm_block
      mask Display: plot(-[0 60 60 55 53 55 60 60 55 53]/150,[0 0 8 16 25 16 8 -8 -16 -25]/50,-[80 80 80 150]/150,[25 -25 0 0]/50,[0 0],[-0.4 0.4],[0.075 0.075],[-0.25 0.25],[0.15 0.15],[-0.1 0.1])
  Sidetruca : PMComponent  Tag=PSATblock  Description=Connection  PhysicalDomain=psatdomain  LeftPortType=p1  RightPortType=p1  LConnTagsString=__newl0  RConnTagsString=__newr0|__newr1  mask(Bus){in=1, out=2, p2q=115, p3_4q=[1.0023    -0.25717], p5q=1, p6q=1}
      mask prompts: in "Number of inputs:"; out "Number of outputs:"; p2q "Voltage Rating [kV]"; p3_4q "Voltage initial guess [p.u.  rad]"; p5q "Area number"; p6q "Region number"
      mask help: Bus block.
      mask init:
      | fm_inout
      settings: AttributesFormatString="|V| =  1.0266 p.u.\\n<V  =  0.0688 rad"
      mask CallbackString: ||||fm_block|
      mask Display: plot([0 1 1 0 0],[0 0 1 1 0])
  Sipororo : PMComponent  Tag=PSATblock  Description=Connection  PhysicalDomain=psatdomain  LeftPortType=p1  RightPortType=p1  LConnTagsString=__newl0|__newl1  RConnTagsString=__newr0  mask(Bus){in=2, out=1, p2q=115, p3_4q=[1.0023    -0.25717], p5q=1, p6q=1}
      mask prompts: in "Number of inputs:"; out "Number of outputs:"; p2q "Voltage Rating [kV]"; p3_4q "Voltage initial guess [p.u.  rad]"; p5q "Area number"; p6q "Region number"
      mask help: Bus block.
      mask init:
      | fm_inout
      settings: AttributesFormatString="|V| =  0.9981 p.u.\\n<V  =  0.0689 rad"
      mask CallbackString: ||||fm_block|
      mask Display: plot([0 1 1 0 0],[0 0 1 1 0])
  Slack : PMComponent  Tag=PSATblock  Description=Power Flow  PhysicalDomain=psatdomain  LeftPortType=p1  RightPortType=p1  RConnTagsString=__newr0  mask(SW){p2_3q=[100  765], p4q=1.04, p5q=0.00, p6_7q=[1.5  -1.5], p8_9q=[1.1  0.9], p10q=30, p11q=1, p12q=on, p13q=on}
      mask prompts: p2_3q "Power and Voltage Ratings [MVA, kV]"; p4q "Voltage Magnitude [p.u.]"; p5q "Reference Phase Angle [rad]"; p6_7q "Qmax and Qmin [p.u.  p.u.]"; p8_9q "Vmax and Vmin  [p.u.  p.u.]"; p10q "Active Power Guess [p.u.]"; p11q "Loss Participation Factor"; p12q "Reference bus"; p13q "Connected"
      mask help:
      | This block defines a V-theta bus:
      |
      | V = V_des
      | theta = theta_des
      mask init:
      | [x,y] = fm_draw('circle');
      | [xt,yt] = fm_draw('theta');
      mask CallbackString: |||||||fm_block|fm_block
      mask Display: plot([0 1 1 0 0],[0 0 1 1 0]), color('blue'), plot([0 1],[0 1],[0 1],[1 0],[0.5 1 0.5 0 0.5],[0 0.5 1 0.5 0])
  Socopo : PMComponent  Tag=PSATblock  Description=Connection  PhysicalDomain=psatdomain  LeftPortType=p1  RightPortType=p1  LConnTagsString=__newl0  RConnTagsString=__newr0|__newr1  mask(Bus){in=1, out=2, p2q=115, p3_4q=[1.0023    -0.25717], p5q=1, p6q=1}
      mask prompts: in "Number of inputs:"; out "Number of outputs:"; p2q "Voltage Rating [kV]"; p3_4q "Voltage initial guess [p.u.  rad]"; p5q "Area number"; p6q "Region number"
      mask help: Bus block.
      mask init:
      | fm_inout
      settings: AttributesFormatString="|V| =  1.0419 p.u.\\n<V  =  0.0989 rad"
      mask CallbackString: ||||fm_block|
      mask Display: plot([0 1 1 0 0],[0 0 1 1 0])
  Sta. Barbara de Barinas : PMComponent  Tag=PSATblock  Description=Connection  PhysicalDomain=psatdomain  LeftPortType=p1  RightPortType=p1  LConnTagsString=__newl0  RConnTagsString=__newr0|__newr1  mask(Bus){in=1, out=2, p2q=115, p3_4q=[1.0023    -0.25717], p5q=1, p6q=1}
      mask prompts: in "Number of inputs:"; out "Number of outputs:"; p2q "Voltage Rating [kV]"; p3_4q "Voltage initial guess [p.u.  rad]"; p5q "Area number"; p6q "Region number"
      mask help: Bus block.
      mask init:
      | fm_inout
      settings: AttributesFormatString="|V| =  0.9937 p.u.\\n<V  =  0.4886 rad"
      mask CallbackString: ||||fm_block|
      mask Display: plot([0 1 1 0 0],[0 0 1 1 0])
  Sur OMZ 230kV : PMComponent  Tag=PSATblock  Description=Connection  PhysicalDomain=psatdomain  LeftPortType=p1  RightPortType=p1  LConnTagsString=__newl0|__newl1|__newl2|__newl3  RConnTagsString=__newr0|__newr1  mask(Bus){in=4, out=2, p2q=230, p3_4q=[1.0224    -0.42388], p5q=1, p6q=1}
      mask prompts: in "Number of inputs:"; out "Number of outputs:"; p2q "Voltage Rating [kV]"; p3_4q "Voltage initial guess [p.u.  rad]"; p5q "Area number"; p6q "Region number"
      mask help: Bus block.
      mask init:
      | fm_inout
      settings: AttributesFormatString="|V| =  1.0312 p.u.\\n<V  = -0.1728 rad"
      mask CallbackString: ||||fm_block|
      mask Display: plot([0 1 1 0 0],[0 0 1 1 0])
  Sur OMZ 765kV : PMComponent  Tag=PSATblock  Description=Connection  PhysicalDomain=psatdomain  LeftPortType=p1  RightPortType=p1  LConnTagsString=__newl0|__newl1  RConnTagsString=__newr0|__newr1  mask(Bus){in=2, out=2, p2q=765, p3_4q=[1.0514    -0.36841], p5q=1, p6q=1}
      mask prompts: in "Number of inputs:"; out "Number of outputs:"; p2q "Voltage Rating [kV]"; p3_4q "Voltage initial guess [p.u.  rad]"; p5q "Area number"; p6q "Region number"
      mask help: Bus block.
      mask init:
      | fm_inout
      settings: AttributesFormatString="|V| =  1.0462 p.u.\\n<V  = -0.1409 rad"
      mask CallbackString: ||||fm_block|
      mask Display: plot([0 1 1 0 0],[0 0 1 1 0])
  Tacoa 230kV : PMComponent  Tag=PSATblock  Description=Connection  PhysicalDomain=psatdomain  LeftPortType=p1  RightPortType=p1  LConnTagsString=__newl0|__newl1|__newl2|__newl3  RConnTagsString=__newr0|__newr1  mask(Bus){in=4, out=2, p2q=230, p3_4q=[1.05    -0.45942], p5q=1, p6q=1}
      mask prompts: in "Number of inputs:"; out "Number of outputs:"; p2q "Voltage Rating [kV]"; p3_4q "Voltage initial guess [p.u.  rad]"; p5q "Area number"; p6q "Region number"
      mask help: Bus block.
      mask init:
      | fm_inout
      settings: AttributesFormatString="|V| =  1.04   p.u.\\n<V  = -0.1946 rad"
      mask CallbackString: ||||fm_block|
      mask Display: plot([0 1 1 0 0],[0 0 1 1 0])
  Termobarrancas 230kV : PMComponent  Tag=PSATblock  Description=Connection  PhysicalDomain=psatdomain  LeftPortType=p1  RightPortType=p1  LConnTagsString=__newl0  RConnTagsString=__newr0  mask(Bus){in=1, out=1, p2q=230, p3_4q=[1.0585     -0.6092], p5q=1, p6q=1}
      mask prompts: in "Number of inputs:"; out "Number of outputs:"; p2q "Voltage Rating [kV]"; p3_4q "Voltage initial guess [p.u.  rad]"; p5q "Area number"; p6q "Region number"
      mask help: Bus block.
      mask init:
      | fm_inout
      settings: AttributesFormatString="|V| =  1.02   p.u.\\n<V  =  0.1213 rad"
      mask CallbackString: ||||fm_block|
      mask Display: plot([0 1 1 0 0],[0 0 1 1 0])
  Tiara 230kV : PMComponent  Tag=PSATblock  Description=Connection  PhysicalDomain=psatdomain  LeftPortType=p1  RightPortType=p1  LConnTagsString=__newl0|__newl1  RConnTagsString=__newr0  mask(Bus){in=2, out=1, p2q=230, p3_4q=[0.95955    -0.48769], p5q=1, p6q=1}
      mask prompts: in "Number of inputs:"; out "Number of outputs:"; p2q "Voltage Rating [kV]"; p3_4q "Voltage initial guess [p.u.  rad]"; p5q "Area number"; p6q "Region number"
      mask help: Bus block.
      mask init:
      | fm_inout
      settings: AttributesFormatString="|V| =  1.0062 p.u.\\n<V  = -0.1858 rad"
      mask CallbackString: ||||fm_block|
      mask Display: plot([0 1 1 0 0],[0 0 1 1 0])
  Tovar : PMComponent  Tag=PSATblock  Description=Connection  PhysicalDomain=psatdomain  LeftPortType=p1  RightPortType=p1  LConnTagsString=__newl0|__newl1  RConnTagsString=__newr0|__newr1|__newr2  mask(Bus){in=2, out=3, p2q=115, p3_4q=[1.0023    -0.25717], p5q=1, p6q=1}
      mask prompts: in "Number of inputs:"; out "Number of outputs:"; p2q "Voltage Rating [kV]"; p3_4q "Voltage initial guess [p.u.  rad]"; p5q "Area number"; p6q "Region number"
      mask help: Bus block.
      mask init:
      | fm_inout
      settings: AttributesFormatString="|V| =  1.004  p.u.\\n<V  =  0.4260 rad"
      mask CallbackString: ||||fm_block|
      mask Display: plot([0 1 1 0 0],[0 0 1 1 0])
  Trinidad 138kV : PMComponent  Tag=PSATblock  Description=Connection  PhysicalDomain=psatdomain  LeftPortType=p1  RightPortType=p1  LConnTagsString=__newl0|__newl1|__newl2  RConnTagsString=__newr0|__newr1  mask(Bus){in=3, out=2, p2q=138, p3_4q=[1.0329    -0.91001], p5q=1, p6q=1}
      mask prompts: in "Number of inputs:"; out "Number of outputs:"; p2q "Voltage Rating [kV]"; p3_4q "Voltage initial guess [p.u.  rad]"; p5q "Area number"; p6q "Region number"
      mask help: Bus block.
      mask init:
      | fm_inout
      settings: AttributesFormatString="|V| =  1.0104 p.u.\\n<V  =  0.0061 rad"
      mask CallbackString: ||||fm_block|
      mask Display: plot([0 1 1 0 0],[0 0 1 1 0])
  Trinidad 230kV : PMComponent  Tag=PSATblock  Description=Connection  PhysicalDomain=psatdomain  LeftPortType=p1  RightPortType=p1  LConnTagsString=__newl0  RConnTagsString=__newr0  mask(Bus){in=1, out=1, p2q=230, p3_4q=[0.99849    -0.84504], p5q=1, p6q=1}
      mask prompts: in "Number of inputs:"; out "Number of outputs:"; p2q "Voltage Rating [kV]"; p3_4q "Voltage initial guess [p.u.  rad]"; p5q "Area number"; p6q "Region number"
      mask help: Bus block.
      mask init:
      | fm_inout
      settings: AttributesFormatString="|V| =  1.0251 p.u.\\n<V  = -0.0181 rad"
      mask CallbackString: ||||fm_block|
      mask Display: plot([0 1 1 0 0],[0 0 1 1 0])
  Trujillo : PMComponent  Tag=PSATblock  Description=Connection  PhysicalDomain=psatdomain  LeftPortType=p1  RightPortType=p1  LConnTagsString=__newl0|__newl1  RConnTagsString=__newr0  mask(Bus){in=2, out=1, p2q=115, p3_4q=[1.0023    -0.25717], p5q=1, p6q=1}
      mask prompts: in "Number of inputs:"; out "Number of outputs:"; p2q "Voltage Rating [kV]"; p3_4q "Voltage initial guess [p.u.  rad]"; p5q "Area number"; p6q "Region number"
      mask help: Bus block.
      mask init:
      | fm_inout
      settings: AttributesFormatString="|V| =  1.0352 p.u.\\n<V  =  0.1067 rad"
      mask CallbackString: ||||fm_block|
      mask Display: plot([0 1 1 0 0],[0 0 1 1 0])
  Turen : PMComponent  Tag=PSATblock  Description=Connection  PhysicalDomain=psatdomain  LeftPortType=p1  RightPortType=p1  LConnTagsString=__newl0|__newl1  RConnTagsString=__newr0  mask(Bus){in=2, out=1, p2q=115, p3_4q=[1.0023    -0.25717], p5q=1, p6q=1}
      mask prompts: in "Number of inputs:"; out "Number of outputs:"; p2q "Voltage Rating [kV]"; p3_4q "Voltage initial guess [p.u.  rad]"; p5q "Area number"; p6q "Region number"
      mask help: Bus block.
      mask init:
      | fm_inout
      settings: AttributesFormatString="|V| =  0.8587 p.u.\\n<V  = -0.1734 rad"
      mask CallbackString: ||||fm_block|
      mask Display: plot([0 1 1 0 0],[0 0 1 1 0])
  Urdaneta 138kV : PMComponent  Tag=PSATblock  Description=Connection  PhysicalDomain=psatdomain  LeftPortType=p1  RightPortType=p1  LConnTagsString=__newl0|__newl1|__newl2  RConnTagsString=__newr0|__newr1  mask(Bus){in=3, out=2, p2q=138, p3_4q=[1.07    -0.87735], p5q=1, p6q=1}
      mask prompts: in "Number of inputs:"; out "Number of outputs:"; p2q "Voltage Rating [kV]"; p3_4q "Voltage initial guess [p.u.  rad]"; p5q "Area number"; p6q "Region number"
      mask help: Bus block.
      mask init:
      | fm_inout
      settings: AttributesFormatString="|V| =  1.04   p.u.\\n<V  =  0.2189 rad"
      mask CallbackString: ||||fm_block|
      mask Display: plot([0 1 1 0 0],[0 0 1 1 0])
  Uribante 115kV : PMComponent  Tag=PSATblock  Description=Connection  PhysicalDomain=psatdomain  LeftPortType=p1  RightPortType=p1  LConnTagsString=__newl0|__newl1|__newl2  RConnTagsString=__newr0  mask(Bus){in=3, out=1, p2q=115, p3_4q=[0.98444    -0.26004], p5q=1, p6q=1}
      mask prompts: in "Number of inputs:"; out "Number of outputs:"; p2q "Voltage Rating [kV]"; p3_4q "Voltage initial guess [p.u.  rad]"; p5q "Area number"; p6q "Region number"
      mask help: Bus block.
      mask init:
      | fm_inout
      settings: AttributesFormatString="|V| =  1.0058 p.u.\\n<V  =  0.5102 rad"
      mask CallbackString: ||||fm_block|
      mask Display: plot([0 1 1 0 0],[0 0 1 1 0])
  Uribante 230kV : PMComponent  Tag=PSATblock  Description=Connection  PhysicalDomain=psatdomain  LeftPortType=p1  RightPortType=p1  LConnTagsString=__newl0|__newl1|__newl2|__newl3|__newl4  RConnTagsString=__newr0|__newr1|__newr2|__newr3  mask(Bus){in=5, out=4, p2q=230, p3_4q=[1.0674    -0.65301], p5q=1, p6q=1}
      mask prompts: in "Number of inputs:"; out "Number of outputs:"; p2q "Voltage Rating [kV]"; p3_4q "Voltage initial guess [p.u.  rad]"; p5q "Area number"; p6q "Region number"
      mask help: Bus block.
      mask init:
      | fm_inout
      settings: AttributesFormatString="|V| =  1.0238 p.u.\\n<V  =  0.5581 rad"
      mask CallbackString: ||||fm_block|
      mask Display: plot([0 1 1 0 0],[0 0 1 1 0])
  Valencia 230kV : PMComponent  Tag=PSATblock  Description=Connection  PhysicalDomain=psatdomain  LeftPortType=p1  RightPortType=p1  LConnTagsString=__newl0  RConnTagsString=__newr0|__newr1|__newr2  mask(Bus){in=1, out=3, p2q=230, p3_4q=[0.94798    -0.58922], p5q=1, p6q=1}
      mask prompts: in "Number of inputs:"; out "Number of outputs:"; p2q "Voltage Rating [kV]"; p3_4q "Voltage initial guess [p.u.  rad]"; p5q "Area number"; p6q "Region number"
      mask help: Bus block.
      mask init:
      | fm_inout
      settings: AttributesFormatString="|V| =  0.9500 p.u.\\n<V  = -0.2296 rad"
      mask CallbackString: ||||fm_block|
      mask Display: plot([0 1 1 0 0],[0 0 1 1 0])
  Valera I : PMComponent  Tag=PSATblock  Description=Connection  PhysicalDomain=psatdomain  LeftPortType=p1  RightPortType=p1  LConnTagsString=__newl0|__newl1  RConnTagsString=__newr0|__newr1  mask(Bus){in=2, out=2, p2q=115, p3_4q=[1.0023    -0.25717], p5q=1, p6q=1}
      mask prompts: in "Number of inputs:"; out "Number of outputs:"; p2q "Voltage Rating [kV]"; p3_4q "Voltage initial guess [p.u.  rad]"; p5q "Area number"; p6q "Region number"
      mask help: Bus block.
      mask init:
      | fm_inout
      settings: AttributesFormatString="|V| =  1.0386 p.u.\\n<V  =  0.1055 rad"
      mask CallbackString: ||||fm_block|
      mask Display: plot([0 1 1 0 0],[0 0 1 1 0])
  Valera II : PMComponent  Tag=PSATblock  Description=Connection  PhysicalDomain=psatdomain  LeftPortType=p1  RightPortType=p1  LConnTagsString=__newl0|__newl1|__newl2|__newl3|__newl4  RConnTagsString=__newr0|__newr1|__newr2|__newr3|__newr4  mask(Bus){in=5, out=5, p2q=115, p3_4q=[0.98444    -0.26004], p5q=1, p6q=1}
      mask prompts: in "Number of inputs:"; out "Number of outputs:"; p2q "Voltage Rating [kV]"; p3_4q "Voltage initial guess [p.u.  rad]"; p5q "Area number"; p6q "Region number"
      mask help: Bus block.
      mask init:
      | fm_inout
      settings: AttributesFormatString="|V| =  1.0363 p.u.\\n<V  =  0.1013 rad"
      mask CallbackString: ||||fm_block|
      mask Display: plot([0 1 1 0 0],[0 0 1 1 0])
  Varname : fm_lib/Connections/Varname  Tag=PSATblock  Description=OPF & CPF  SystemSampleTime=-1  pxq="[55  62  66  73  94  100  111  166  173  177  184  205  211  222]"
  Vueltosa 230kV : PMComponent  Tag=PSATblock  Description=Connection  PhysicalDomain=psatdomain  LeftPortType=p1  RightPortType=p1  LConnTagsString=__newl0  RConnTagsString=__newr0|__newr1  mask(Bus){in=1, out=2, p2q=230, p3_4q=[1 0], p5q=1, p6q=1}
      mask prompts: in "Number of inputs:"; out "Number of outputs:"; p2q "Voltage Rating [kV]"; p3_4q "Voltage initial guess [p.u.  rad]"; p5q "Area number"; p6q "Region number"
      mask help: Bus block.
      mask init:
      | fm_inout
      settings: AttributesFormatString="|V| =  1.02   p.u.\\n<V  =  0.5759 rad"
      mask CallbackString: ||||fm_block|
      mask Display: plot([0 1 1 0 0],[0 0 1 1 0])
  Yaracuy 230kV : PMComponent  Tag=PSATblock  Description=Connection  PhysicalDomain=psatdomain  LeftPortType=p1  RightPortType=p1  LConnTagsString=__newl0|__newl1|__newl2|__newl3  RConnTagsString=__newr0|__newr1|__newr2|__newr3|__newr4|__newr5  mask(Bus){in=4, out=6, p2q=230, p3_4q=[0.9567      -0.546], p5q=1, p6q=1}
      mask prompts: in "Number of inputs:"; out "Number of outputs:"; p2q "Voltage Rating [kV]"; p3_4q "Voltage initial guess [p.u.  rad]"; p5q "Area number"; p6q "Region number"
      mask help: Bus block.
      mask init:
      | fm_inout
      settings: AttributesFormatString="|V| =  0.9550 p.u.\\n<V  = -0.1363 rad"
      mask CallbackString: ||||fm_block|
      mask Display: plot([0 1 1 0 0],[0 0 1 1 0])
  Yaracuy 400kV : PMComponent  Tag=PSATblock  Description=Connection  PhysicalDomain=psatdomain  LeftPortType=p1  RightPortType=p1  LConnTagsString=__newl0|__newl1|__newl2|__newl3  RConnTagsString=__newr0|__newr1|__newr2|__newr3  mask(Bus){in=4, out=4, p2q=400, p3_4q=[0.94273    -0.52379], p5q=1, p6q=1}
      mask prompts: in "Number of inputs:"; out "Number of outputs:"; p2q "Voltage Rating [kV]"; p3_4q "Voltage initial guess [p.u.  rad]"; p5q "Area number"; p6q "Region number"
      mask help: Bus block.
      mask init:
      | fm_inout
      settings: AttributesFormatString="|V| =  0.9771 p.u.\\n<V  = -0.1204 rad"
      mask CallbackString: ||||fm_block|
      mask Display: plot([0 1 1 0 0],[0 0 1 1 0])
  Yaracuy 765kV : PMComponent  Tag=PSATblock  Description=Connection  PhysicalDomain=psatdomain  LeftPortType=p1  RightPortType=p1  LConnTagsString=__newl0|__newl1|__newl2  RConnTagsString=__newr0|__newr1|__newr2|__newr3  mask(Bus){in=3, out=4, p2q=765, p3_4q=[0.98704    -0.46859], p5q=1, p6q=1}
      mask prompts: in "Number of inputs:"; out "Number of outputs:"; p2q "Voltage Rating [kV]"; p3_4q "Voltage initial guess [p.u.  rad]"; p5q "Area number"; p6q "Region number"
      mask help: Bus block.
      mask init:
      | fm_inout
      settings: AttributesFormatString="|V| =  0.9339 p.u.\\n<V  = -0.1363 rad"
      mask CallbackString: ||||fm_block|
      mask Display: plot([0 1 1 0 0],[0 0 1 1 0])
  connections:
  Guri 765kV/LConn6 -- Auto15/LConn1
  Guri 765kV/LConn5 -- Auto1/LConn1
  Guri 765kV/LConn4 -- Auto2/LConn1
  Auto3/RConn1 -- Guri 230kV/LConn1
  El Tigre 400kV/LConn1 -- Line22/LConn1
  El Tigre 400kV/LConn2 -- Line27/LConn1
  La Canoa 400kV/LConn1 -- Line17/LConn1
  La Canoa 400kV/LConn2 -- Line16/RConn1
  Auto4/RConn1 -- San Geronimo 400kV/LConn1
  Auto5/RConn1 -- San Geronimo 400kV/LConn2
  El Tigre 400kV/LConn3 -- Auto7/LConn1
  El Tigre 400kV/LConn4 -- Auto6/LConn1
  Line6/RConn1 -- Macagua II/LConn3
  Guayana B/LConn1 -- Line9/LConn1
  Guayana B/LConn2 -- Line47/LConn1
  Line9/RConn1 -- Macagua II/LConn1
  Line47/RConn1 -- Macagua II/LConn2
  Line105/LConn1 -- Guri 230kV/LConn3
  Line19/LConn1 -- Guri 230kV/LConn2
  Line152/RConn1 -- Ciudad Bolivar 230kV/RConn1
  Line36/RConn1 -- Ciudad Bolivar 230kV/LConn1
  Malena 765kV/LConn1 -- Line3/RConn1
  Malena 765kV/LConn2 -- Line4/RConn1
  Malena 765kV/LConn3 -- Line5/RConn1
  San Geronimo 765kV/LConn5 -- Auto4/LConn1
  San Geronimo 765kV/LConn4 -- Auto5/LConn1
  Guri 400kV B/LConn1 -- Auto15/RConn1
  Guri 400kV B/LConn2 -- Auto1/RConn1
  Guri 400kV B/LConn3 -- Auto2/RConn1
  Guri 400kV A/LConn6 -- Auto3/LConn1
  Guri 400kV A/LConn5 -- Line7/LConn1
  Guri 400kV A/LConn4 -- Line101/LConn1
  Guri 400kV A/LConn3 -- Line18/LConn1
  Guri 400kV A/LConn2 -- Line16/LConn1
  Guri 400kV B/LConn4 -- Auto16/LConn1
  Auto16/RConn1 -- Guri 400kV A/LConn1
  Line144/LConn1 -- Guri 400kV B/RConn3
  Line157/RConn1 -- Guri 400kV B/RConn1
  Line15/RConn1 -- Guri 400kV B/RConn2
  Guayana B/RConn1 -- Line15/LConn1
  Guayana B/RConn2 -- Line157/LConn1
  Line8/LConn1 -- Guayana B/LConn3
  Line19/RConn1 -- Guayana A/RConn1
  Line105/RConn1 -- Guayana A/RConn2
  Guayana A/LConn1 -- Line152/LConn1
  El Tigre 230kV/LConn6 -- Line36/LConn1
  El Tigre 230kV/LConn5 -- Line25/LConn1
  Line56/LConn1 -- Guayana A/LConn2
  Line56/RConn1 -- Ciudad Bolivar 230kV/RConn2
  Ciudad Bolivar 230kV/LConn2 -- Line25/RConn1
  Auto6/RConn1 -- El Tigre 230kV/RConn3
  Auto7/RConn1 -- El Tigre 230kV/RConn2
  PQ46/LConn1 -- Malena 765kV/RConn1
  PQ68/LConn1 -- El Tigre 230kV/RConn4
  Slack/RConn1 -- Guri 765kV/RConn1
  PQ32/LConn1 -- Ciudad Bolivar 230kV/RConn3
  PQ29/LConn1 -- Guayana A/LConn4
  Line27/RConn1 -- San Geronimo 400kV/RConn3
  Line22/RConn1 -- San Geronimo 400kV/RConn2
  PQ28/LConn1 -- San Geronimo 400kV/RConn1
  PQ34/LConn1 -- El Tigre 230kV/RConn1
  Guayana B/LConn4 -- PQ36/LConn1
  PV12/RConn1 -- Guayana A/LConn3
  PV9/RConn1 -- Guri 400kV A/RConn1
  Caruachi/LConn2 -- PV11/RConn1
  PV8/RConn1 -- Guri 230kV/RConn1
  Macagua II/RConn2 -- PV14/RConn1
  PQ43/LConn1 -- San Geronimo 765kV/RConn6
  SC1/RConn1 -- San Geronimo 765kV/RConn5
  Line5/LConn1 -- San Geronimo 765kV/RConn4
  Line4/LConn1 -- San Geronimo 765kV/RConn3
  Line3/LConn1 -- San Geronimo 765kV/RConn2
  Guri 765kV/LConn1 -- Line/RConn1
  Guri 765kV/LConn2 -- Line1/RConn1
  Guri 765kV/LConn3 -- Line2/RConn1
  Line101/RConn1 -- El Tigre 400kV/RConn4
  Line18/RConn1 -- El Tigre 400kV/RConn3
  Line17/RConn1 -- El Tigre 400kV/RConn2
  Line183/RConn1 -- El Tigre 400kV/RConn1
  Line183/LConn1 -- Gen. Anz 2012-2/RConn1
  Line13/LConn1 -- Furrial 400kV/LConn1
  Line7/RConn1 -- Palital 400kV/RConn2
  Palital 400kV/LConn1 -- Line13/RConn1
  Line8/RConn1 -- Palital 400kV/RConn1
  Palital 400kV/LConn2 -- Line73/RConn1
  Line73/LConn1 -- Furrial 400kV/LConn2
  Auto73/LConn1 -- Furrial 400kV/RConn1
  Auto73/RConn1 -- Furrial 230kV/RConn3
  Furrial 230kV/RConn2 -- Line99/LConn1
  Furrial 230kV/RConn1 -- Line30/LConn1
  Furrial 400kV/RConn2 -- PQ12/LConn1
  Palital 400kV/LConn3 -- PQ31/LConn1
  El Tigre 230kV/LConn1 -- Line31/LConn1
  El Tigre 230kV/LConn2 -- Line28/LConn1
  Line146/LConn1 -- El Tigre 400kV/LConn5
  Jose 400kV/LConn2 -- Line23/RConn1
  San Geronimo 400kV/LConn3 -- Line23/LConn1
  El Tigre 230kV/LConn3 -- Line74/LConn1
  El Tigre 230kV/LConn4 -- Line34/LConn1
  Line34/RConn1 -- Furrial 230kV/LConn2
  Line74/RConn1 -- Furrial 230kV/LConn1
  Line146/RConn1 -- Barbacoa II 400kV/LConn2
  Barbacoa II 400kV/RConn1 -- Auto11/LConn1
  Jose 400kV/LConn1 -- Line147/LConn1
  Line147/RConn1 -- Barbacoa II 400kV/LConn1
  Barbacoa II 230kV/RConn1 -- Auto11/RConn1
  Santa Teresa 400kV/RConn1 -- Line35/RConn1
  Line20/RConn1 -- Santa Teresa 400kV/RConn2
  Line20/LConn1 -- San Geronimo 400kV/LConn5
  Ciudad Losada 400kV/LConn1 -- Line38/LConn1
  Line38/RConn1 -- Santa Teresa 400kV/RConn3
  Auto20/RConn1 -- Santa Teresa 230kV/LConn2
  Auto18/RConn1 -- Santa Teresa 230kV/LConn1
  Sur OMZ 765kV/LConn1 -- Auto22/LConn1
  Sur OMZ 765kV/LConn2 -- Auto19/LConn1
  Auto22/RConn1 -- Sur OMZ 230kV/RConn1
  Auto19/RConn1 -- Sur OMZ 230kV/RConn2
  Santa Teresa 400kV/LConn1 -- Auto20/LConn1
  Santa Teresa 400kV/LConn2 -- Auto18/LConn1
  Line39/LConn1 -- Sur OMZ 765kV/RConn2
  Line40/LConn1 -- Sur OMZ 765kV/RConn1
  Sur OMZ 230kV/LConn4 -- Line14/LConn1
  Sur OMZ 230kV/LConn3 -- Line26/LConn1
  Line26/RConn1 -- Papelon 230kV/RConn1
  Line14/RConn1 -- Papelon 230kV/RConn2
  Line46/RConn1 -- Junquito 230kV/RConn1
  Line10/RConn1 -- Junquito 230kV/RConn2
  Line10/LConn1 -- Sur OMZ 230kV/LConn2
  Sur OMZ 230kV/LConn1 -- Line46/LConn1
  Santa Teresa 230kV/LConn3 -- Line164/LConn1
  Line164/RConn1 -- Papelon 230kV/RConn3
  Santa Teresa 230kV/LConn4 -- Line50/LConn1
  Line48/RConn1 -- Papelon 230kV/LConn1
  Line45/RConn1 -- Boyaca 230kV/LConn1
  Line54/RConn1 -- Convento 230kV/LConn1
  Line53/RConn1 -- Convento 230kV/LConn2
  Junquito 230kV/LConn3 -- Line48/LConn1
  Boyaca 230kV/LConn2 -- Line54/LConn1
  Line50/RConn1 -- Convento 230kV/LConn3
  Auto21/RConn1 -- La Horqueta 230kV/LConn1
  Auto17/RConn1 -- Ciudad Losada 230kV/LConn1
  Ciudad Losada 230kV/RConn2 -- Line66/LConn1
  Ciudad Losada 230kV/RConn1 -- Line63/LConn1
  Line67/RConn1 -- La Horqueta 230kV/RConn4
  Line158/RConn1 -- Santa Teresa 230kV/RConn1
  Line21/RConn1 -- Santa Teresa 230kV/RConn2
  Line33/RConn1 -- Santa Teresa 230kV/RConn4
  Line32/RConn1 -- Santa Teresa 230kV/RConn3
  Barbacoa II 230kV/LConn2 -- Line24/LConn1
  Barbacoa II 230kV/LConn1 -- Line72/LConn1
  Rio Chico II/LConn1 -- Line37/LConn1
  Rio Chico II/RConn1 -- Line33/LConn1
  Line28/RConn1 -- Barbacoa I 230kV/LConn3
  Line31/RConn1 -- Barbacoa I 230kV/LConn2
  Barbacoa II 230kV/LConn3 -- Line55/LConn1
  Line29/LConn1 -- Barbacoa II 230kV/LConn4
  Line66/RConn1 -- La Horqueta 230kV/RConn5
  Auto26/RConn1 -- La Horqueta 230kV/RConn1
  Auto25/RConn1 -- La Horqueta 230kV/LConn2
  La Horqueta 230kV/LConn5 -- Line76/LConn1
  La Horqueta 230kV/LConn6 -- Line80/LConn1
  La Horqueta 230kV/LConn7 -- Line78/LConn1
  La Horqueta 230kV/LConn8 -- Line98/LConn1
  Line98/RConn1 -- Macaro 230kV/RConn2
  Line78/RConn1 -- Macaro 230kV/RConn1
  Line82/RConn1 -- Macaro 230kV/LConn1
  Macaro 230kV/LConn2 -- Line81/RConn1
  San Geronimo 765kV/LConn3 -- Line39/RConn1
  Ciudad Losada 230kV/LConn3 -- Line158/LConn1
  Ciudad Losada 230kV/LConn2 -- Line21/LConn1
  PQ61/LConn1 -- Santa Teresa 400kV/RConn4
  Santa Teresa 230kV/RConn5 -- Line71/LConn1
  Line71/RConn1 -- Barbacoa I 230kV/RConn1
  Line37/RConn1 -- Barbacoa I 230kV/RConn2
  Line72/RConn1 -- Barbacoa I 230kV/RConn3
  Line24/RConn1 -- Barbacoa I 230kV/RConn4
  Junquito 230kV/LConn1 -- Line52/LConn1
  Line52/RConn1 -- Tacoa 230kV/RConn1
  Macaro 230kV/LConn3 -- PQ22/LConn1
  Junquito 230kV/LConn2 -- PQ39/LConn1
  PQ41/LConn1 -- Tacoa 230kV/RConn2
  PQ42/LConn1 -- Boyaca 230kV/RConn1
  PQ44/LConn1 -- Convento 230kV/RConn1
  Papelon 230kV/LConn2 -- PQ40/LConn1
  Rio Chico II/LConn2 -- PQ14/LConn1
  Ciudad Losada 230kV/LConn4 -- PQ26/LConn1
  Tacoa 230kV/LConn1 -- PV2/RConn1
  Santa Teresa 230kV/LConn5 -- PQ27/LConn1
  San Geronimo 400kV/LConn4 -- Line35/LConn1
  PQ33/LConn1 -- Jose 400kV/RConn1
  Barbacoa I 230kV/LConn1 -- PQ13/LConn1
  Tacoa 230kV/LConn4 -- Line45/LConn1
  Tacoa 230kV/LConn3 -- Line53/LConn1
  Santa Teresa 230kV/LConn6 -- Line179/LConn1
  Line179/RConn1 -- Gen. Miranda 2012/RConn1
  Jose 400kV/RConn2 -- Line182/RConn1
  Gen. Anz 2012-1/RConn1 -- Line182/LConn1
  La Horqueta 765kV/RConn3 -- Line40/RConn1
  Line140/LConn1 -- La Horqueta 765kV/RConn1
  Line44/LConn1 -- La Horqueta 765kV/RConn2
  Auto23/LConn1 -- La Horqueta 765kV/LConn1
  Auto26/LConn1 -- La Horqueta 765kV/LConn2
  Line140/RConn1 -- La Arenosa 765kV/RConn4
  Ciudad Losada 400kV/RConn1 -- Auto17/LConn1
  Tiara 230kV/LConn2 -- Line63/RConn1
  Tiara 230kV/LConn1 -- Line67/LConn1
  La Arenosa 765kV/LConn1 -- Auto28/LConn1
  La Arenosa 765kV/LConn2 -- Auto24/LConn1
  Auto23/RConn1 -- La Horqueta 400kV/RConn2
  Line77/RConn1 -- La Horqueta 230kV/LConn3
  Line89/RConn1 -- La Horqueta 230kV/LConn4
  Aragua 230kV/LConn2 -- Line76/RConn1
  Aragua 230kV/LConn1 -- Line80/RConn1
  Line79/RConn1 -- Aragua 230kV/RConn2
  Caña de Azucar 230kV/LConn2 -- Line82/LConn1
  Caña de Azucar 230kV/LConn1 -- Line83/RConn1
  La Horqueta 400kV/LConn4 -- Auto21/LConn1
  La Horqueta 400kV/LConn3 -- Auto25/LConn1
  Line64/RConn1 -- La Horqueta 400kV/LConn2
  Line70/RConn1 -- La Horqueta 400kV/LConn1
  San Diego 230kV/LConn4 -- Line83/LConn1
  San Diego 230kV/LConn3 -- Line81/LConn1
  La Arenosa 400kV/LConn6 -- Auto29/LConn1
  La Arenosa 400kV/LConn5 -- Line64/LConn1
  La Arenosa 400kV/LConn4 -- Line70/LConn1
  Line87/RConn1 -- San Diego 230kV/LConn1
  Line94/RConn1 -- San Diego 230kV/LConn2
  Auto29/RConn1 -- La Arenosa 230kV/LConn1
  San Geronimo 765kV/LConn2 -- Line44/RConn1
  La Arenosa 230kV/RConn5 -- Line110/RConn1
  La Arenosa 230kV/RConn7 -- Line94/LConn1
  La Arenosa 230kV/RConn6 -- Line87/LConn1
  Auto28/RConn1 -- La Arenosa 230kV/RConn1
  Auto24/RConn1 -- La Arenosa 230kV/RConn2
  La Arenosa 230kV/LConn8 -- Line79/LConn1
  La Arenosa 230kV/LConn7 -- Line65/LConn1
  La Arenosa 230kV/LConn6 -- Line77/LConn1
  La Arenosa 230kV/LConn5 -- Line89/LConn1
  Line88/LConn1 -- La Arenosa 230kV/LConn4
  Line86/LConn1 -- La Arenosa 230kV/LConn3
  PQ4/LConn1 -- La Arenosa 765kV/RConn5
  La Horqueta 400kV/RConn1 -- PQ65/LConn1
  La Arenosa 400kV/RConn1 -- PQ66/LConn1
  La Horqueta 765kV/RConn4 -- SC3/RConn1
  Aragua 230kV/RConn3 -- Line32/LConn1
  PQ21/LConn1 -- Caña de Azucar 230kV/RConn1
  PQ18/LConn1 -- La Arenosa 230kV/RConn8
  PQ19/LConn1 -- San Diego 230kV/RConn1
  Aragua 230kV/LConn3 -- PQ20/LConn1
  Line108/RConn1 -- La Horqueta 230kV/RConn3
  Line107/RConn1 -- La Horqueta 230kV/RConn2
  San Fernando II 230kV/LConn1 -- Line109/LConn1
  PQ25/LConn1 -- San Fernando II 230kV/RConn1
  PV13/RConn1 -- San Diego 230kV/RConn2
  Line65/RConn1 -- Aragua 230kV/RConn1
  PQ17/LConn1 -- Valencia 230kV/LConn1
  San Geronimo 765kV/LConn1 -- Line43/RConn1
  Line43/LConn1 -- La Arenosa 765kV/RConn3
  Line109/RConn1 -- Calabozo 230kV/RConn1
  Calabozo 230kV/LConn3 -- Line108/LConn1
  Calabozo 230kV/LConn2 -- Line107/LConn1
  Line88/RConn1 -- Valencia 230kV/RConn3
  Line86/RConn1 -- Valencia 230kV/RConn2
  PQ24/LConn1 -- Calabozo 230kV/RConn3
  Line174/LConn1 -- San Fernando II 230kV/LConn2
  Line174/RConn1 -- Calabozo 230kV/RConn2
  Line178/RConn1 -- Calabozo 230kV/LConn1
  Line178/LConn1 -- Gen. Guarico 2012/RConn1
  PV6/RConn1 -- Guanta II 230kV/RConn1
  Guanta II 230kV/LConn1 -- Auto9/LConn1
  Auto9/RConn1 -- Guanta II 115kV/RConn1
  Guanta II 115kV/LConn1 -- Line154/RConn1
  Guanta II 115kV/LConn2 -- Line162/RConn1
  Guanta II 230kV/LConn2 -- PQ69/LConn1
  Line29/RConn1 -- Guanta II 230kV/RConn4
  Line55/RConn1 -- Guanta II 230kV/RConn3
  Cumana III/LConn2 -- Line165/LConn1
  Cumana III/LConn1 -- Line166/RConn1
  PQ71/LConn1 -- Cumana III/RConn1
  El Indio 230kV/LConn2 -- Line100/LConn1
  El Indio 230kV/LConn1 -- Line155/LConn1
  Line30/RConn1 -- El Indio 230kV/RConn1
  Line99/RConn1 -- El Indio 230kV/RConn2
  Line155/RConn1 -- Casanay 230kV/RConn3
  Line100/RConn1 -- Casanay 230kV/RConn4
  Casanay 230kV/RConn2 -- Line75/RConn1
  Casanay 230kV/RConn1 -- Line151/RConn1
  PQ59/LConn1 -- El Indio 230kV/RConn3
  PQ35/LConn1 -- El Indio 230kV/LConn3
  Line162/LConn1 -- Cumana II/LConn3
  Line154/LConn1 -- Cumana II/LConn2
  Guanta II 230kV/LConn4 -- Line75/LConn1
  Guanta II 230kV/LConn3 -- Line151/LConn1
  Line165/RConn1 -- Cumana II/LConn1
  Line166/LConn1 -- Manzanares/LConn1
  Cumana II/RConn1 -- Line167/RConn1
  Line167/LConn1 -- Manzanares/LConn2
  Casanay 230kV/LConn1 -- Auto8/LConn1
  Auto8/RConn1 -- Casanay 115kV/LConn1
  Cariaco/LConn1 -- Line168/RConn1
  Cumana II/RConn2 -- Line169/RConn1
  Line169/LConn1 -- Cariaco/RConn1
  Line168/LConn1 -- Casanay 115kV/RConn2
  Cumana II/RConn3 -- Line170/RConn1
  Line170/LConn1 -- Casanay 115kV/RConn1
  PQ57/LConn1 -- Cumana II/RConn4
  Manzanares/RConn1 -- PQ70/LConn1
  Cariaco/LConn2 -- PQ72/LConn1
  PQ47/LConn1 -- Casanay 115kV/LConn2
  Gen. Miranda 2012/LConn1 -- PV15/RConn1
  PV16/RConn1 -- Gen. Anz 2012-2/LConn1
  PV17/RConn1 -- Gen. Anz 2012-1/LConn1
  Gen. Guarico 2012/LConn1 -- PV18/RConn1
  Casanay 115kV/RConn3 -- Line171/RConn1
  Casanay 115kV/RConn4 -- Line172/RConn1
  Chicopata/LConn1 -- Line171/LConn1
  Line172/LConn1 -- Chicopata/LConn2
  Chicopata/RConn1 -- Line156/RConn1
  Luisa Caceres/LConn3 -- PQ73/LConn1
  Luisa Caceres/LConn2 -- PV/RConn1
  Line156/LConn1 -- Luisa Caceres/RConn2
  Line11/RConn1 -- El Callao II 400kV/RConn1
  Macagua II/RConn1 -- Line11/LConn1
  Auto66/RConn1 -- Las Claritas 230kV/RConn1
  Auto66/LConn1 -- Las Claritas 400kV/LConn2
  Las Claritas 400kV/RConn1 -- Line12/RConn1
  Line12/LConn1 -- El Callao II 400kV/RConn2
  Las Claritas 230kV/LConn1 -- Line148/LConn1
  PQ67/LConn1 -- Las Claritas 400kV/LConn1
  El Callao II 400kV/LConn1 -- PQ30/LConn1
  Line148/RConn1 -- Santa Elena/RConn1
  Santa Elena/LConn1 -- Line149/LConn1
  Line149/RConn1 -- Boa Vista (Brasil)/RConn1
  PQ60/LConn1 -- Santa Elena/LConn2
  PQ1/LConn1 -- Boa Vista (Brasil)/LConn1
  PV10/RConn1 -- Urdaneta 138kV/RConn1
  PV5/RConn1 -- Ramon Laguna 138kV/RConn1
  La Arenosa 400kV/RConn2 -- Line95/RConn1
  Line41/LConn1 -- La Arenosa 765kV/RConn1
  Auto37/RConn1 -- Planta Centro 230kV/LConn1
  La Arenosa 230kV/RConn3 -- Line92/LConn1
  La Arenosa 230kV/RConn4 -- Line163/LConn1
  Yaracuy 765kV/LConn1 -- Auto38/LConn1
  Yaracuy 765kV/LConn2 -- Auto39/LConn1
  Auto38/RConn1 -- Yaracuy 400kV/RConn4
  Auto39/RConn1 -- Yaracuy 230kV/RConn1
  Yaracuy 400kV/LConn4 -- Auto40/LConn1
  Auto40/RConn1 -- Yaracuy 230kV/LConn1
  Line95/LConn1 -- Yaracuy 400kV/RConn3
  Yaracuy 400kV/RConn2 -- Line91/LConn1
  La Arenosa 400kV/LConn2 -- Line85/LConn1
  La Arenosa 400kV/LConn1 -- Line90/LConn1
  Line106/RConn1 -- Cabudare 230kV/RConn2
  Line96/RConn1 -- Cabudare 230kV/RConn3
  Line84/RConn1 -- Yaracuy 230kV/RConn6
  Line122/RConn1 -- Yaracuy 230kV/RConn5
  Auto72/RConn1 -- Yaracuy 230kV/RConn2
  Yaracuy 765kV/LConn3 -- Auto72/LConn1
  La Arenosa 230kV/LConn2 -- Line93/LConn1
  PQ62/LConn1 -- Yaracuy 400kV/RConn1
  Cabudare 230kV/LConn1 -- Line110/LConn1
  PQ45/LConn1 -- Planta Centro 230kV/RConn6
  Yaracuy 230kV/LConn2 -- Line106/LConn1
  Yaracuy 230kV/LConn3 -- Line96/LConn1
  Yaracuy 230kV/LConn4 -- PQ49/LConn1
  PQ16/LConn1 -- Cabudare 230kV/RConn1
  Line93/RConn1 -- Planta Centro 230kV/RConn5
  Line92/RConn1 -- Planta Centro 230kV/RConn4
  Line163/RConn1 -- Planta Centro 230kV/RConn3
  PQ2/LConn1 -- Yaracuy 765kV/RConn2
  Yaracuy 765kV/RConn4 -- Line41/RConn1
  Yaracuy 765kV/RConn3 -- Line42/RConn1
  Planta Centro 400kV/LConn1 -- PV7/RConn1
  Line42/LConn1 -- La Arenosa 765kV/RConn2
  PQ54/LConn1 -- P. Piedra 138kV/LConn1
  Line127/RConn1 -- P. Iguana/RConn1
  P. Iguana/LConn1 -- Line133/RConn1
  PQ37/LConn1 -- Cuatricentenario 138kV/LConn1
  P. Piedra 230kV/RConn1 -- Line133/LConn1
  Auto27/RConn1 -- P. Piedra 138kV/RConn1
  P. Piedra 230kV/LConn1 -- Auto27/LConn1
  El Rincon 138kV/LConn2 -- PQ53/LConn1
  PQ55/LConn1 -- Urdaneta 138kV/LConn3
  Line135/RConn1 -- Urdaneta 138kV/LConn1
  Line136/RConn1 -- Urdaneta 138kV/LConn2
  El Rincon 138kV/LConn1 -- Line139/RConn1
  Auto30/RConn1 -- El Rincon 138kV/RConn1
  Line104/RConn1 -- Morochas 230kV/RConn4
  Line103/RConn1 -- Morochas 230kV/RConn3
  Line102/RConn1 -- Morochas 230kV/RConn2
  Line103/LConn1 -- Yaracuy 230kV/RConn4
  Yaracuy 230kV/RConn3 -- Line104/LConn1
  PQ58/LConn1 -- Morochas 230kV/RConn1
  Shunt2/LConn1 -- Morochas 230kV/RConn5
  Yaracuy 400kV/LConn3 -- Line60/LConn1
  Line59/LConn1 -- Yaracuy 400kV/LConn2
  Line97/LConn1 -- Yaracuy 400kV/LConn1
  Auto49/RConn1 -- El Tablazo 230kV/LConn1
  Line113/RConn1 -- El Tablazo 230kV/RConn1
  El Tablazo 400kV/LConn3 -- Auto49/LConn1
  El Tablazo 400kV/LConn1 -- Line123/LConn1
  El Tablazo 400kV/LConn2 -- Line49/LConn1
  El Tablazo 230kV/LConn2 -- Line126/LConn1
  El Tablazo 230kV/LConn3 -- Line58/LConn1
  Line126/RConn1 -- P. Palmas/RConn1
  Line58/RConn1 -- P. Palmas/RConn2
  P. Palmas/LConn1 -- Line129/RConn1
  P. Palmas/LConn2 -- Line57/RConn1
  Line114/RConn1 -- Cabimas 230kV/RConn2
  Cabimas 230kV/RConn1 -- Line112/LConn1
  El Tablazo 230kV/RConn2 -- Line112/RConn1
  PQ63/LConn1 -- El Tablazo 400kV/RConn1
  El Tablazo 230kV/LConn4 -- Line127/LConn1
  PQ5/LConn1 -- El Tablazo 230kV/LConn5
  Line97/RConn1 -- El Tablazo 400kV/RConn2
  Line59/RConn1 -- El Tablazo 400kV/RConn3
  Line60/RConn1 -- El Tablazo 400kV/RConn4
  Auto56/RConn1 -- Cuatricentenario 230kV/LConn1
  Line123/RConn1 -- Cuatricentenario 400kV/RConn1
  Line49/RConn1 -- Cuatricentenario 400kV/RConn2
  Peonias/LConn1 -- Line125/LConn1
  Cuatricentenario 230kV/RConn1 -- Line125/RConn1
  Cuatricentenario 230kV/RConn2 -- Line51/RConn1
  Line51/LConn1 -- Peonias/LConn2
  Line129/LConn1 -- Peonias/RConn1
  Line57/LConn1 -- Peonias/RConn2
  Cuatricentenario 400kV/LConn1 -- Auto56/LConn1
  Cuestecita (Colombia)/LConn1 -- Line138/LConn1
  Auto60/RConn1 -- Cuatricentenario 138kV/RConn1
  Cuatricentenario 230kV/LConn5 -- Auto60/LConn1
  Cuatricentenario 230kV/LConn4 -- Line134/LConn1
  Cuatricentenario 230kV/LConn3 -- Line131/LConn1
  Line138/RConn1 -- Cuatricentenario 230kV/LConn2
  El Rincon 138kV/RConn3 -- Line128/LConn1
  Line128/RConn1 -- Ramon Laguna 138kV/LConn4
  Trinidad 138kV/RConn2 -- Line137/LConn1
  Auto31/RConn1 -- Trinidad 138kV/RConn1
  Trinidad 138kV/LConn3 -- Line139/LConn1
  Trinidad 230kV/LConn1 -- Auto31/LConn1
  El Rincon 230kV/LConn1 -- Auto30/LConn1
  Line137/RConn1 -- Ramon Laguna 138kV/LConn2
  PQ52/LConn1 -- Trinidad 138kV/LConn1
  Line130/RConn1 -- Ramon Laguna 138kV/LConn5
  P. Piedra 138kV/RConn2 -- Line130/LConn1
  Line132/RConn1 -- Trinidad 138kV/LConn2
  Line131/RConn1 -- Trinidad 230kV/RConn1
  Line124/LConn1 -- El Rincon 138kV/RConn2
  Line134/RConn1 -- El Rincon 230kV/RConn1
  Line124/RConn1 -- Ramon Laguna 138kV/LConn3
  Cuatricentenario 138kV/RConn2 -- Line132/LConn1
  PQ51/LConn1 -- Ramon Laguna 138kV/LConn1
  Termobarrancas 230kV/LConn1 -- Line161/LConn1
  Line161/RConn1 -- Barinas IV 230kV/RConn1
  Las Flores 230kV/LConn1 -- Line143/LConn1
  Line68/RConn1 -- Barinas IV 230kV/LConn1
  Barinas IV 230kV/LConn2 -- Line141/RConn1
  Barinas IV 230kV/LConn3 -- Line120/LConn1
  Line120/RConn1 -- Las Flores 230kV/RConn1
  Line118/RConn1 -- Planta Paez 230kV/RConn1
  Uribante 230kV/LConn3 -- Line116/LConn1
  Line116/RConn1 -- San Agaton 230kV/RConn1
  Uribante 230kV/LConn4 -- Line61/LConn1
  Line61/RConn1 -- San Agaton 230kV/RConn2
  Line160/RConn1 -- Uribante 230kV/RConn1
  Line69/RConn1 -- Uribante 230kV/RConn2
  Line141/LConn1 -- Planta Paez 230kV/RConn3
  Line68/LConn1 -- Planta Paez 230kV/RConn2
  PV3/RConn1 -- Planta Paez 230kV/LConn1
  PV4/RConn1 -- San Agaton 230kV/LConn1
  Shunt4/LConn1 -- El Corozo 230kV/RConn4
  El Corozo 230kV/LConn1 -- Line160/LConn1
  El Corozo 230kV/LConn2 -- Line69/LConn1
  Line115/RConn1 -- El Corozo 230kV/RConn3
  Line111/RConn1 -- El Corozo 230kV/RConn2
  Buena Vista 230kV/LConn1 -- Line102/LConn1
  Line62/RConn1 -- Buena Vista 230kV/RConn1
  El Vigia II 230kV/LConn1 -- Line62/LConn1
  Line118/LConn1 -- Buena Vista 230kV/RConn2
  San Mateo 230kV/RConn1 -- Line111/LConn1
  San Mateo 230kV/RConn2 -- Line115/LConn1
  PQ48/LConn1 -- San Mateo 230kV/LConn1
  PV22/RConn1 -- Termobarrancas 230kV/RConn1
  Acarigua II 230kV/LConn1 -- Line122/LConn1
  Acarigua II 230kV/LConn2 -- Line84/LConn1
  Line143/RConn1 -- Acarigua II 230kV/RConn1
  Acarigua II 230kV/RConn2 -- Line159/RConn1
  Barinas IV 230kV/LConn4 -- Line159/LConn1
  Line119/RConn1 -- Planta Centro 230kV/RConn1
  Line121/RConn1 -- Planta Centro 230kV/RConn2
  Isiro 230kV/RConn1 -- Auto50/LConn1
  PQ64/LConn1 -- Isiro 230kV/RConn2
  Isiro 230kV/LConn1 -- Line119/LConn1
  Isiro 230kV/LConn2 -- Line121/LConn1
  Auto50/RConn1 -- Isiro 115kV/RConn1
  Isiro 115kV/LConn4 -- PQ50/LConn1
  Isiro 115kV/LConn3 -- Line145/LConn1
  Line145/RConn1 -- Coro II/RConn1
  Punto Fijo II/LConn2 -- Line153/LConn1
  Punto Fijo II/LConn1 -- Line150/LConn1
  Line150/RConn1 -- Punto Fijo I/LConn1
  Line153/RConn1 -- Punto Fijo I/LConn2
  Punto Fijo I/RConn1 -- PV1/RConn1
  PQ56/LConn1 -- Punto Fijo II/RConn3
  Line142/RConn1 -- Punto Fijo II/RConn2
  Line173/RConn1 -- Punto Fijo II/RConn1
  Isiro 115kV/LConn1 -- Line173/LConn1
  Isiro 115kV/LConn2 -- Line142/LConn1
  Coro II/LConn2 -- Shunt3/LConn1
  PV38/RConn1 -- Coro II/LConn1
  Vueltosa 230kV/LConn1 -- PV19/RConn1
  Uribante 230kV/RConn3 -- Line175/LConn1
  Gen. Zulia 2012/LConn1 -- PV20/RConn1
  Cabimas 230kV/LConn1 -- Line176/LConn1
  Line176/RConn1 -- Gen. Zulia 2012/RConn1
  Line2/LConn1 -- Malena 765kV/RConn4
  Line1/LConn1 -- Malena 765kV/RConn3
  Line/LConn1 -- Malena 765kV/RConn2
  El Rincon 138kV/RConn5 -- Line136/LConn1
  El Rincon 138kV/RConn4 -- Line135/LConn1
  Planta Centro 400kV/LConn3 -- Auto37/LConn1
  Line85/RConn1 -- Planta Centro 400kV/RConn3
  Line91/RConn1 -- Planta Centro 400kV/RConn1
  Line90/RConn1 -- Planta Centro 400kV/RConn2
  Line144/RConn1 -- Caruachi/RConn1
  Caruachi/LConn1 -- Line6/LConn1
  Line177/RConn1 -- Uribante 230kV/LConn1
  Line177/LConn1 -- El Vigia II 230kV/RConn1
  Line175/RConn1 -- Vueltosa 230kV/RConn2
  Line117/LConn1 -- El Vigia II 230kV/RConn2
  Line117/RConn1 -- Uribante 230kV/LConn2
  Line114/LConn1 -- Morochas 230kV/LConn1
  Morochas 230kV/LConn2 -- Line113/LConn1
  PQ8/LConn1 -- Uribante 115kV/LConn1
  Uribante 230kV/LConn5 -- Auto43/LConn1
  Auto43/RConn1 -- Uribante 115kV/RConn1
  Uribante 115kV/LConn2 -- Line211/LConn1
  Line210/LConn1 -- Uribante 115kV/LConn3
  Sta. Barbara de Barinas/RConn1 -- Line210/RConn1
  PQ110/LConn1 -- Sta. Barbara de Barinas/RConn2
  La Pedrera/RConn1 -- Line211/RConn1
  PQ111/LConn1 -- La Pedrera/LConn1
  La Pedrera/RConn2 -- Line209/LConn1
  Sta. Barbara de Barinas/LConn1 -- Line208/LConn1
  Line208/RConn1 -- Guasdualito/RConn1
  Line209/RConn1 -- Guasdualito/RConn2
  Guasdualito/LConn3 -- PQ113/LConn1
  Guasdualito/LConn2 -- Line280/LConn1
  Guasdualito/LConn1 -- Line279/LConn1
  Elorza/RConn1 -- Line280/RConn1
  Elorza/RConn2 -- Line279/RConn1
  PQ112/LConn1 -- Elorza/LConn1
  Barinas IV 230kV/LConn5 -- Auto45/LConn1
  Auto45/RConn1 -- Barinas IV 115kV/RConn1
  PQ117/LConn1 -- Barinas IV 115kV/LConn1
  Barinas IV 115kV/LConn2 -- Line207/LConn1
  Line207/RConn1 -- Socopo/LConn1
  Socopo/RConn2 -- Shunt11/LConn1
  Socopo/RConn1 -- PQ114/LConn1
  Acarigua II 115kV/LConn3 -- PQ10/LConn1
  Line190/RConn1 -- Acarigua II 115kV/LConn1
  Turen/RConn1 -- Line190/LConn1
  PQ121/LConn1 -- Turen/LConn1
  Line191/RConn1 -- Turen/LConn2
  El Playon/RConn1 -- Line191/LConn1
  PQ123/LConn1 -- El Playon/LConn1
  Acarigua II 230kV/LConn3 -- Auto47/LConn1
  Auto47/RConn1 -- Acarigua II 115kV/RConn1
  Acarigua II 115kV/RConn4 -- Line187/LConn1
  Acarigua II 115kV/RConn3 -- Line186/LConn1
  Line187/RConn1 -- Acarigua I/RConn1
  Line186/RConn1 -- Acarigua I/RConn2
  PQ125/LConn1 -- Acarigua I/LConn2
  Shunt18/LConn1 -- Acarigua I/LConn1
  Acarigua II 115kV/LConn2 -- Line192/RConn1
  Line192/LConn1 -- Araure/LConn1
  Araure/LConn2 -- Line194/LConn1
  PQ124/LConn1 -- Araure/RConn1
  PQ122/LConn1 -- Guanare/LConn2
  Shunt17/LConn1 -- Guanare/LConn3
  Guanare/RConn1 -- Line194/RConn1
  Guanare/RConn3 -- Line193/LConn1
  Line193/RConn1 -- Acarigua I/LConn3
  Las Flores 230kV/LConn2 -- Auto46/LConn1
  Las Flores 115kV/RConn1 -- Auto46/RConn1
  PQ11/LConn1 -- Las Flores 115kV/LConn1
  Las Flores 115kV/RConn2 -- Line195/LConn1
  Line195/RConn1 -- Guanare/RConn2
  Line197/RConn1 -- Guanare/LConn1
  Pena Larga/LConn1 -- Line197/LConn1
  PV21/RConn1 -- Pena Larga/RConn1
  Pena Larga/LConn2 -- Line281/LConn1
  Shunt16/LConn1 -- Barinas II/RConn2
  Barinas II/LConn1 -- Line202/LConn1
  Barinas II/LConn2 -- PQ119/LConn1
  Line202/RConn1 -- Barinas III/LConn1
  Barinas III/RConn1 -- PQ120/LConn1
  Barinas III/LConn2 -- Line203/LConn1
  Barinas I/RConn1 -- Line203/RConn1
  Barinas I/RConn3 -- PV24/RConn1
  Barinas I/RConn4 -- PQ118/LConn1
  Masparro/LConn1 -- Line281/RConn1
  PV29/RConn1 -- Masparro/RConn1
  Masparro/LConn2 -- Line198/RConn1
  Line198/LConn1 -- Barinas I/LConn6
  Barinas IV 115kV/RConn2 -- Line201/LConn1
  Barinas IV 115kV/RConn3 -- Line200/LConn1
  Barinas IV 115kV/RConn4 -- Line282/LConn1
  Line201/RConn1 -- Barinas II/RConn1
  Line282/RConn1 -- Barinas I/LConn5
  Line200/RConn1 -- Barinas I/LConn4
  Line196/RConn1 -- Sipororo/RConn1
  Line196/LConn1 -- Las Flores 115kV/LConn2
  Sipororo/LConn1 -- Line199/LConn1
  Sipororo/LConn2 -- PQ3/LConn1
  Line199/RConn1 -- Barinas I/LConn1
  Barinas I/RConn2 -- Line204/LConn1
  El Torereno/LConn1 -- Line204/RConn1
  El Torereno/LConn2 -- PQ116/LConn1
  Line205/LConn1 -- El Torereno/RConn1
  Shunt12/LConn1 -- El Torereno/RConn2
  La Libertad/LConn1 -- Line205/RConn1
  PQ115/LConn1 -- La Libertad/RConn1
  Shunt15/LConn1 -- La Libertad/RConn2
  El Corozo 230kV/RConn1 -- Auto44/LConn1
  Auto44/RConn1 -- El Corozo 115kV/LConn4
  El Corozo 115kV/RConn5 -- PQ15/LConn1
  El Corozo 115kV/RConn4 -- Line278/RConn1
  El Corozo 115kV/RConn3 -- Line188/LConn1
  La Concordia/RConn1 -- Line278/LConn1
  La Concordia/RConn2 -- Line188/RConn1
  PQ103/LConn1 -- La Concordia/LConn1
  El Corozo 115kV/RConn1 -- Line216/RConn1
  San Cristobal I/LConn2 -- Shunt14/LConn1
  Line216/LConn1 -- San Cristobal I/RConn2
  San Cristobal I/LConn1 -- PQ107/LConn1
  Shunt10/LConn1 -- San Antonio/LConn2
  San Antonio/RConn2 -- PQ109/LConn1
  San Antonio/RConn1 -- Line231/RConn1
  El Corozo 115kV/RConn2 -- Line231/LConn1
  Mucubaji/LConn1 -- Line212/RConn1
  Line212/LConn1 -- Planta Paez 115kV/LConn3
  Line206/RConn1 -- Planta Paez 115kV/LConn4
  Line283/RConn1 -- Planta Paez 115kV/LConn5
  Planta Paez 115kV/RConn4 -- PV25/RConn1
  PQ9/LConn1 -- Planta Paez 115kV/LConn1
  Planta Paez 230kV/LConn3 -- Auto10/LConn1
  Auto10/RConn1 -- Planta Paez 115kV/RConn1
  PQ100/LConn1 -- Mucubaji/RConn2
  Line283/LConn1 -- Barinas I/LConn2
  Barinas I/LConn3 -- Line206/LConn1
  Shunt8/LConn1 -- Merida II/LConn3
  Merida II/RConn4 -- PQ102/LConn1
  Merida I/RConn1 -- Line215/RConn1
  Merida I/RConn2 -- PQ101/LConn1
  Shunt9/LConn1 -- Merida I/LConn1
  Merida II/RConn3 -- Line215/LConn1
  Merida II/RConn2 -- Line214/RConn1
  Merida II/RConn1 -- Line213/RConn1
  Line214/LConn1 -- Mucubaji/RConn1
  Planta Paez 115kV/LConn2 -- Line213/LConn1
  PQ104/LConn1 -- Palo Grande/RConn2
  Palo Grande/LConn1 -- Line228/RConn1
  Line228/LConn1 -- El Corozo 115kV/LConn3
  El Corozo 115kV/LConn2 -- Line227/LConn1
  Line227/RConn1 -- San Cristobal II/LConn1
  PQ106/LConn1 -- San Cristobal II/RConn2
  Line230/LConn1 -- Palo Grande/RConn1
  Line230/RConn1 -- Planta Tachira/RConn4
  Planta Tachira/RConn3 -- Line229/RConn1
  Line229/LConn1 -- San Cristobal II/RConn1
  PQ108/LConn1 -- Planta Tachira/LConn4
  PV27/RConn1 -- Planta Tachira/LConn1
  Planta Tachira/RConn1 -- Line219/LConn1
  Planta Tachira/RConn2 -- Line220/LConn1
  Line219/RConn1 -- La Grita/LConn1
  Line220/RConn1 -- La Grita/LConn2
  Line221/RConn1 -- La Grita/LConn3
  PQ99/LConn1 -- La Grita/LConn4
  Line221/LConn1 -- El Corozo 115kV/LConn1
  Line218/LConn1 -- San Cristobal I/RConn1
  Line218/RConn1 -- La Grita/RConn3
  La Fria II/RConn4 -- PQ105/LConn1
  La Fria II/RConn2 -- Line234/LConn1
  La Fria II/RConn1 -- Line233/LConn1
  Line234/RConn1 -- Planta Tachira/LConn3
  Line233/RConn1 -- Planta Tachira/LConn2
  Line232/LConn1 -- San Antonio/LConn1
  Line232/RConn1 -- La Fria II/RConn3
  La Fria II/LConn1 -- Line235/LConn1
  Line235/RConn1 -- El Vigia/LConn1
  PQ96/LConn1 -- El Vigia/LConn2
  El Vigia/RConn4 -- Shunt7/LConn1
  El Vigia/RConn3 -- Line224/RConn1
  Line223/RConn1 -- La Grita/RConn2
  La Grita/RConn1 -- Line222/RConn1
  Line223/LConn1 -- Tovar/RConn3
  Line222/LConn1 -- Tovar/RConn2
  Line224/LConn1 -- Tovar/RConn1
  Tovar/LConn2 -- PQ97/LConn1
  PQ98/LConn1 -- Ejido/RConn2
  Line217/RConn1 -- Tovar/LConn1
  Line217/LConn1 -- Ejido/RConn1
  Ejido/LConn1 -- Line225/RConn1
  Line225/LConn1 -- Merida II/LConn2
  El Vigia/RConn2 -- Line226/RConn1
  Line226/LConn1 -- Merida II/LConn1
  Auto12/RConn1 -- El Vigia II 115kV/RConn1
  El Vigia II 230kV/LConn2 -- Auto12/LConn1
  PQ6/LConn1 -- El Vigia II 115kV/LConn3
  El Vigia/RConn1 -- Line236/LConn1
  Line236/RConn1 -- El Vigia II 115kV/LConn2
  San Carlos del Zulia/LConn2 -- PQ95/LConn1
  PV26/RConn1 -- San Carlos del Zulia/RConn1
  San Carlos del Zulia/LConn1 -- Line237/RConn1
  Line237/LConn1 -- El Vigia II 115kV/LConn1
  Shunt13/LConn1 -- Caja Seca/RConn1
  PQ85/LConn1 -- Caja Seca/RConn2
  Caja Seca/LConn1 -- Line238/RConn1
  Line238/LConn1 -- Buena Vista 115kV/LConn2
  PQ23/LConn1 -- Buena Vista 115kV/LConn1
  Buena Vista 230kV/LConn2 -- Auto13/LConn1
  Auto13/RConn1 -- Buena Vista 115kV/RConn1
  Buena Vista 115kV/RConn2 -- Line256/RConn1
  Buena Vista 115kV/RConn3 -- Line259/RConn1
  Buena Vista 115kV/RConn4 -- Line260/RConn1
  Line259/LConn1 -- Valera I/LConn1
  PQ86/LConn1 -- Valera I/LConn2
  Shunt19/LConn1 -- Valera I/RConn2
  Valera I/RConn1 -- Line189/LConn1
  Line189/RConn1 -- Valera II/LConn5
  Shunt1/LConn1 -- Valera II/RConn5
  PQ78/LConn1 -- Valera II/RConn4
  Valera II/LConn1 -- Line239/RConn1
  Line239/LConn1 -- Trujillo/RConn1
  Trujillo/LConn2 -- PQ92/LConn1
  Trujillo/LConn1 -- Line260/LConn1
  Valera II/LConn4 -- Line256/LConn1
  Valera II/LConn3 -- Line255/RConn1
  Valera II/LConn2 -- Line254/RConn1
  Line255/LConn1 -- Planta Paez 115kV/RConn2
  Line254/LConn1 -- Planta Paez 115kV/RConn3
  PQ74/LConn1 -- Cemento Andino/RConn1
  Cemento Andino/LConn1 -- Line245/RConn1
  Line245/LConn1 -- Monay/RConn1
  Monay/LConn2 -- PQ38/LConn1
  Monay/LConn1 -- Line251/RConn1
  Valera II/RConn3 -- Line251/LConn1
  PQ76/LConn1 -- Sidetruca/RConn1
  Sidetruca/RConn2 -- Line240/RConn1
  Line240/LConn1 -- Valera II/RConn2
  Valera II/RConn1 -- Line241/RConn1
  Sidetruca/LConn1 -- Line244/RConn1
  PQ75/LConn1 -- San Lorenzo/RConn2
  PV30/RConn1 -- San Lorenzo/RConn1
  San Lorenzo/LConn4 -- Line244/LConn1
  San Lorenzo/LConn3 -- Line241/LConn1
  San Lorenzo/LConn1 -- Line252/RConn1
  Line252/LConn1 -- Machango/RConn1
  PQ77/LConn1 -- Machango/RConn2
  Machango/LConn1 -- Line253/RConn1
  Line253/LConn1 -- Puricaure/LConn1
  Puricaure/RConn1 -- PQ79/LConn1
  San Lorenzo/LConn2 -- Line261/RConn1
  Line261/LConn1 -- Morochas 115kV/LConn2
  Morochas 230kV/LConn3 -- Auto14/LConn1
  Auto14/RConn1 -- Morochas 115kV/RConn1
  PQ7/LConn1 -- Morochas 115kV/LConn1
  PQ80/LConn1 -- Cabimas 230kV/LConn2
  Morochas 115kV/RConn2 -- PV23/RConn1
  Acarigua I/RConn3 -- PV28/RConn1
